simulink model "PreCondition"  (R2018b)
settings: Solver=FixedStepDiscrete  StartTime=0.0  StopTime=10.0  FixedStep=0.01  RelTol=1e-3
undefined symbols (not defined in the file or in its folder): EnergyMgLdShdRq1, HMI_2L_StMd10_Config_Val, HMI_2L_StMd11_Config_Val, HMI_2L_StMd12_Config_Val, HMI_2L_StMd13_Config_Val, HMI_2L_StMd14_Config_Val, HMI_2L_StMd15_Config_Val, HMI_2L_StMd16_Config_Val, HMI_2L_StMd17_Config_Val, HMI_2L_StMd18_Config_Val, HMI_2L_StMd19_Config_Val, HMI_2L_StMd1_Config_Val, HMI_2L_StMd20_Config_Val, HMI_2L_StMd21_Config_Val, HMI_2L_StMd22_Config_Val, HMI_2L_StMd23_Config_Val, HMI_2L_StMd24_Config_Val, HMI_2L_StMd25_Config_Val, HMI_2L_StMd26_Config_Val, HMI_2L_StMd27_Config_Val, HMI_2L_StMd28_Config_Val, HMI_2L_StMd29_Config_Val, HMI_2L_StMd2_Config_Val, HMI_2L_StMd30_Config_Val, HMI_2L_StMd31_Config_Val, HMI_2L_StMd32_Config_Val, HMI_2L_StMd3_Config_Val, HMI_2L_StMd4_Config_Val, HMI_2L_StMd5_Config_Val, HMI_2L_StMd6_Config_Val, HMI_2L_StMd7_Config_Val, HMI_2L_StMd8_Config_Val, HMI_2L_StMd9_Config_Val, HMI_2R_StMd10_Config_Val, HMI_2R_StMd11_Config_Val, HMI_2R_StMd12_Config_Val, HMI_2R_StMd13_Config_Val, HMI_2R_StMd14_Config_Val, HMI_2R_StMd15_Config_Val, HMI_2R_StMd16_Config_Val, HMI_2R_StMd17_Config_Val, HMI_2R_StMd18_Config_Val, HMI_2R_StMd19_Config_Val, HMI_2R_StMd1_Config_Val, HMI_2R_StMd20_Config_Val, HMI_2R_StMd21_Config_Val, HMI_2R_StMd22_Config_Val, HMI_2R_StMd23_Config_Val, HMI_2R_StMd24_Config_Val, HMI_2R_StMd25_Config_Val, HMI_2R_StMd26_Config_Val, HMI_2R_StMd27_Config_Val, HMI_2R_StMd28_Config_Val, HMI_2R_StMd29_Config_Val, HMI_2R_StMd2_Config_Val, HMI_2R_StMd30_Config_Val, HMI_2R_StMd31_Config_Val, HMI_2R_StMd32_Config_Val, HMI_2R_StMd3_Config_Val, HMI_2R_StMd4_Config_Val ... (+94)
(part 4 of 6)

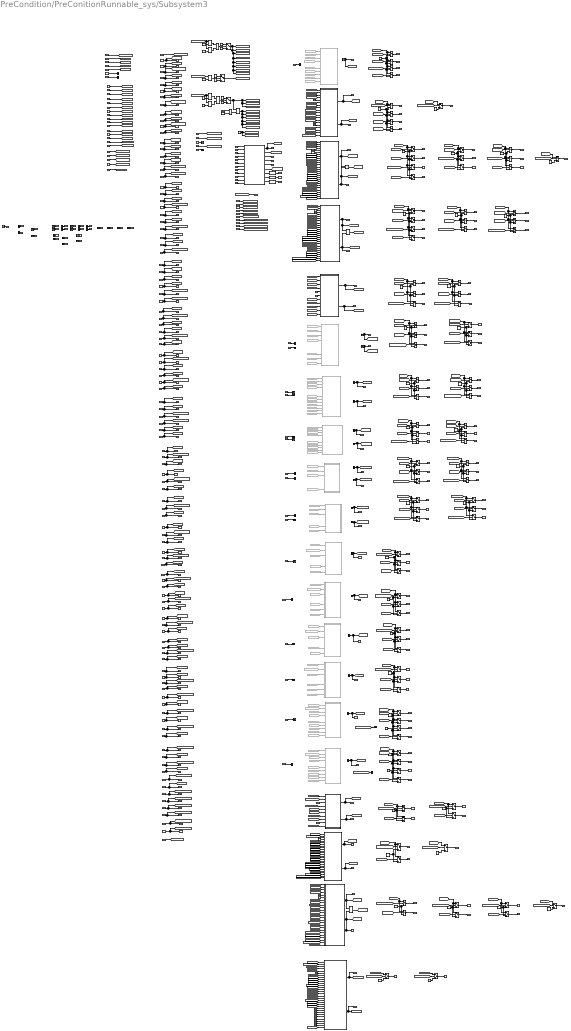
== system PreCondition/PreConitionRunnable_sys/Subsystem3 ==
  note: #大四座的前提条件和AcsEntry一致
  note: NOTE:
      | 2023-08-01:
      | 1.新增mode21~26的前提条件更改，REQ_MSM_778
      | 2.增加PSM,vip或者全躺模式/腿托一键打开增加位置前后判断，REQ_MSM_631/787/788
      | 2023-11-27：
      | 1.腿托一键打开，VIP功能，全躺功能不限制座椅前后位置
      | 2.增加诊断C02C
  note: 4座不包含亲密模式，照看模式
  note: #LyingR
  note: #LyingL
  note: #RcvyR
  note: #VipR
  note: #RcvyL
  note: #VIpL
  note: #LuggageR
  note: #LuggageL
  note: #Family—2R
  note: #Intimacy
  note: #Luggage All
  note: #VIP All
  note: //13，14提供给扶手屏
  note: //2，3提供给扶手屏
  note: #Family—2L
  note: #LgrstOpenLt
  note: #LgrstCloseLt
  note: #LgrstOpenRt
  note: #LgrstCloseRt
  note: #VIPAllOut
  note: #ExVIPR的前提条件和VIPR一致
  SysPwrMd : Inport
  SysPwrMdV : Inport  Port=2
  VoltSts : Inport  Port=3
  EnergyMgLdShdRq : Inport  Port=4
  MmryRclImpctDisRq : Inport  Port=5
  AbgDplyBckp : Inport  Port=6
  AbgDplyBckpV : Inport  Port=7
  VehMovState : Inport  Port=8
  VehSpdAvgDrvnV : Inport  Port=9
  VehSpdAvgDrvn : Inport  Port=10
  DrvStPosRclRspStat : Inport  Port=11
  PassStPosRclRspStat : Inport  Port=12
  SecRwLtStPosRclRspStat : Inport  Port=13
  SecRwRtStPosRclRspStat : Inport  Port=14
  ThdRwLtStPosRclRspStat : Inport  Port=15
  ThdRwRtStPosRclRspStat : Inport  Port=16
  AcsEntryPosLrnd : Inport  Port=17
  AcsExitPosLrnd : Inport  Port=18
  VIPLtPosLrnd : Inport  Port=19
  VIPRtPosLrnd : Inport  Port=20
  LugLtPosLrnd : Inport  Port=21
  LugRtPosLrnd : Inport  Port=22
  RcvyLtPosLrnd : Inport  Port=23
  RcvyRtPosLrnd : Inport  Port=24
  ThdRwLtStOccStatMSMSrc : Inport  Port=25
  ThdRwCtStOccStatMSMSrc : Inport  Port=26
  ThdRwRtStOccStatMSMSrc : Inport  Port=27
  SecRwLtStChldLkReq : Inport  Port=28
  SecRwRtStChldLkReq : Inport  Port=29
  IsDrvStSwAct : Inport  Port=30
  IsPasStSwAct : Inport  Port=31
  Is2LStSwAct : Inport  Port=32
  Is2RStSwAct : Inport  Port=33
  Is3LStSwAct : Inport  Port=34
  Is3RStSwAct : Inport  Port=35
  VeSignalLost2R_463_2L : Inport  Port=36
  VeSignalLost3L_468_2L : Inport  Port=37
  "VeSignalLost3R_46C_2L " : Inport  Port=38
  VeSignalLostCODR_470_2L : Inport  Port=39
  VeSignalLostDR_213_2L : Inport  Port=40
  KeSMSbRoofSWEnable : Inport  Port=41
  VeSignalLostSDM_195_2L : Inport  Port=42
  VeSignalLostFireWall_1D2_2L : Inport  Port=43
  IntimacyLPosLrnd : Inport  Port=44
  IntimacyRPosLrnd : Inport  Port=45
  FamilyLtPosLrnd : Inport  Port=46
  FamilyRtPosLrnd : Inport  Port=47
  LyingLtPosLrnd : Inport  Port=48
  LyingRtPosLrnd : Inport  Port=49
  HMI_2L_StMd1_Config : Inport  Port=50
  HMI_2R_StMd1_Config : Inport  Port=51
  StPassCmprtMdCtrl_Md1_VCUConfig : Inport  Port=52
  StSrv_StMd1_Config : Inport  Port=53
  HMI_2L_StMd2_Config : Inport  Port=54
  HMI_2R_StMd2_Config : Inport  Port=55
  StPassCmprtMdCtrl_Md2_VCUConfig : Inport  Port=56
  StSrv_StMd2_Config : Inport  Port=57
  HMI_2L_StMd10_Config : Inport  Port=58
  HMI_2R_StMd12_Config : Inport  Port=59
  StSrv_StMd10_Config : Inport  Port=60
  StSrv_StMd12_Config : Inport  Port=61
  StPassCmprtMdCtrl_Md10_VCUConfig : Inport  Port=62
  StPassCmprtMdCtrl_Md12_VCUConfig : Inport  Port=63
  HMI_2L_StMd4_Config : Inport  Port=64
  HMI_2R_StMd4_Config : Inport  Port=65
  StSrv_StMd4_Config : Inport  Port=66
  StPassCmprtMdCtrl_Md4_VCUConfig : Inport  Port=67
  HMI_2L_StMd3_Config : Inport  Port=68
  HMI_2R_StMd3_Config : Inport  Port=69
  StSrv_StMd3_Config : Inport  Port=70
  StPassCmprtMdCtrl_Md3_VCUConfig : Inport  Port=71
  HMI_2L_StMd8_Config : Inport  Port=72
  HMI_2R_StMd9_Config : Inport  Port=73
  StSrv_StMd8_Config : Inport  Port=74
  StPassCmprtMdCtrl_Md8_VCUConfig : Inport  Port=75
  StSrv_StMd9_Config : Inport  Port=76
  StPassCmprtMdCtrl_Md9_VCUConfig : Inport  Port=77
  HMI_2L_StMd11_Config : Inport  Port=78
  HMI_2R_StMd13_Config : Inport  Port=79
  StSrv_StMd11_Config : Inport  Port=80
  StSrv_StMd13_Config : Inport  Port=81
  StPassCmprtMdCtrl_Md11_VCUConfig : Inport  Port=82
  StPassCmprtMdCtrl_Md13_VCUConfig : Inport  Port=83
  HMI_2L_StMd5_Config : Inport  Port=84
  HMI_2R_StMd20_Config : Inport  Port=85
  StPassCmprtMdCtrl_Md5_VCUConfig : Inport  Port=86
  StPassCmprtMdCtrl_Md20_VCUConfig : Inport  Port=87
  StSrv_StMd5_Config : Inport  Port=88
  StSrv_StMd20_Config : Inport  Port=89
  HMI_2R_StMd6_Config : Inport  Port=90
  HMI_2L_StMd7_Config : Inport  Port=91
  StPassCmprtMdCtrl_Md6_VCUConfig : Inport  Port=92
  StSrv_StMd6_Config : Inport  Port=93
  StPassCmprtMdCtrl_Md7_VCUConfig : Inport  Port=94
  StSrv_StMd7_Config : Inport  Port=95
  HMI_2L_StMd14_Config : Inport  Port=96
  HMI_2R_StMd15_Config : Inport  Port=97
  StPassCmprtMdCtrl_Md14_VCUConfig : Inport  Port=98
  StPassCmprtMdCtrl_Md15_VCUConfig : Inport  Port=99
  StSrv_StMd14_Config : Inport  Port=100
  StSrv_StMd15_Config : Inport  Port=101
  LgrstOpenLtPosLrnd : Inport  Port=102
  LgrstCloseLtPosLrnd : Inport  Port=103
  LgrstOpenRtPosLrnd : Inport  Port=104
  LgrstCloseRtPosLrnd : Inport  Port=105
  HMI_2L_StMd16_Config : Inport  Port=106
  StPassCmprtMdCtrl_Md16_VCUConfig : Inport  Port=107
  StSrv_StMd16_Config : Inport  Port=108
  HMI_2L_StMd17_Config : Inport  Port=109
  StPassCmprtMdCtrl_Md17_VCUConfig : Inport  Port=110
  StSrv_StMd17_Config : Inport  Port=111
  HMI_2R_StMd18_Config : Inport  Port=112
  StPassCmprtMdCtrl_Md18_VCUConfig : Inport  Port=113
  StSrv_StMd18_Config : Inport  Port=114
  HMI_2R_StMd19_Config : Inport  Port=115
  StPassCmprtMdCtrl_Md19_VCUConfig : Inport  Port=116
  StSrv_StMd19_Config : Inport  Port=117
  IfVeSMSeStNumConfig : Inport  Port=118
  KeSMSLegrstDisFwdBkwdPos : Inport  Port=119
  SecRwLtStFrwdBkwdPos : Inport  Port=120
  "SecRwLtStFrwdBkwdPosV " : Inport  Port=121
  "SecRwRtStFrwdBkwdPos " : Inport  Port=122
  "SecRwRtStFrwdBkwdPosV " : Inport  Port=123
  AcsEntry4s2LPosLrnd : Inport  Port=124
  HMI_2L_StMd21_Config : Inport  Port=125
  StPassCmprtMdCtrl_Md21_VCUConfig : Inport  Port=126
  StSrv_StMd21_Config : Inport  Port=127
  AcsEntry4s2RPosLrnd : Inport  Port=128
  HMI_2R_StMd23_Config : Inport  Port=129
  StPassCmprtMdCtrl_Md23_VCUConfig : Inport  Port=130
  StSrv_StMd23_Config : Inport  Port=131
  AcsExit4s2LPosLrnd : Inport  Port=132
  HMI_2L_StMd22_Config : Inport  Port=133
  StPassCmprtMdCtrl_Md22_VCUConfig : Inport  Port=134
  StSrv_StMd22_Config : Inport  Port=135
  AcsExit4s2RPosLrnd : Inport  Port=136
  HMI_2R_StMd24_Config : Inport  Port=137
  StPassCmprtMdCtrl_Md24_VCUConfig : Inport  Port=138
  StSrv_StMd24_Config : Inport  Port=139
  AcsEntryAll4sFwdPosLrnd : Inport  Port=140
  HMI_2L_StMd26_Config : Inport  Port=141
  HMI_2R_StMd26_Config : Inport  Port=142
  StPassCmprtMdCtrl_Md26_VCUConfig : Inport  Port=143
  StSrv_StMd26_Config : Inport  Port=144
  AcsEntryAll4sBwdPosLrnd : Inport  Port=145
  HMI_2L_StMd25_Config : Inport  Port=146
  HMI_2R_StMd25_Config : Inport  Port=147
  StPassCmprtMdCtrl_Md25_VCUConfig : Inport  Port=148
  StSrv_StMd25_Config : Inport  Port=149
  IfKeSMSbSeatMovFrwdBkwdEnable : Inport  Port=150
  PassReclinerPosLrnd : Inport  Port=151
  unfold3LPosLrnd : Inport  Port=152
  unfold3RPosLrnd : Inport  Port=153
  NotCoDrvStOccStatBDFSrc : Inport  Port=154
  StPassCmprtMdCtrl_Md30_VCUConfig : Inport  Port=155
  StSrv_StMd30_Config : Inport  Port=156
  StPassCmprtMdCtrl_Md31_VCUConfig : Inport  Port=157
  StSrv_StMd31_Config : Inport  Port=158
  StPassCmprtMdCtrl_Md32_VCUConfig : Inport  Port=159
  StSrv_StMd32_Config : Inport  Port=160
  VIPLtOutPosLrnd : Inport  Port=161
  VIPRtOutPosLrnd : Inport  Port=162
  StPassCmprtMdCtrl_Md27_VCUConfig : Inport  Port=163
  StSrv_StMd27_Config : Inport  Port=164
  StPassCmprtMdCtrl_Md28_VCUConfig : Inport  Port=165
  StSrv_StMd28_Config : Inport  Port=166
  StPassCmprtMdCtrl_Md29_VCUConfig : Inport  Port=167
  StSrv_StMd29_Config : Inport  Port=168
  ThdRwLtStCshnFldUpwdDnwdPos : Inport  Port=169
  ThdRwLtStCshnFldUpwdDnwdPosV : Inport  Port=170
  ThdRwRtStCshnFldUpwdDnwdPos : Inport  Port=171
  ThdRwRtStCshnFldUpwdDnwdPosV : Inport  Port=172
  ThdRwLtStChldLkReq : Inport  Port=173
  NotSecRowLeStOccStatBDFSrc : Inport  Port=174
  NotSecRowRtStOccStatBDFSrc : Inport  Port=175
  SecRwLtStBkReclnUpwdDnwdPos : Inport  Port=176
  SecRwLtStBkReclnUpwdDnwdPosV : Inport  Port=177
  SecRwRtStBkReclnUpwdDnwdPos : Inport  Port=178
  SecRwRtStBkReclnUpwdDnwdPosV : Inport  Port=179
  KeSMSuSecRwStBackPosDelta : Inport  Port=180
  StPassCmprtMdCtrl_Md53_VCUConfig : Inport  Port=181
  StPassCmprtMdCtrl_Md56_VCUConfig : Inport  Port=182
  KeSMSuThrdRwCushFoldPosThreshold : Inport  Port=183
  StPassCmprtMdCtrl_Md57_VCUConfig : Inport  Port=184
  StPassCmprtMdCtrl_Md58_VCUConfig : Inport  Port=185
  PasReclinerPosAvail : Inport  Port=186
  KeSMSwAcsMd32SecRwLtStBkReclnUpwdDnwdPos1 : Inport  Port=187
  KeSMSwAcsMd53SecRwRtStBkReclnUpwdDnwdPos1 : Inport  Port=188
  KeSMSwAcsMd8SecRwLtStBkReclnUpwdDnwdPos : Inport  Port=189
  KeSMSwAcsMd9SecRwRtStBkReclnUpwdDnwdPos : Inport  Port=190
  WholeVehMemPosLrnd : Inport  Port=191
  StPassCmprtMdCtrl_Md61_VCUConfig : Inport  Port=192
  StPassCmprtMdCtrl_Md62_VCUConfig : Inport  Port=193
  KeSMSwSeatBkLimitPos : Inport  Port=194
  KeSMSwSeatBkLimitPosDelt : Inport  Port=195
  Md61PassStBkReclnTrgtPos : Inport  Port=196
  Md61ThdRwLtStCshnFldUpwdDnwdTrgtPos : Inport  Port=197
  Md61ThdRwRtStCshnFldUpwdDnwdTrgtPos : Inport  Port=198
  Md62PassStBkReclnTrgtPos : Inport  Port=199
  Md62ThdRwLtStCshnFldUpwdDnwdTrgtPos : Inport  Port=200
  Md62ThdRwRtStCshnFldUpwdDnwdTrgtPos : Inport  Port=201
  KeSMSuThrdRwCushFoldPosDelta : Inport  Port=202
  AND{,1..3,5} (5 alike) : Logic  Operator=OR  AllPortsSameDT=off  OutDataTypeStr=boolean
  AND4 : Logic  AllPortsSameDT=off  OutDataTypeStr=boolean
  AcsEntry4s2LMd : Subsystem  Commented=on
  AcsEntry4s2RMd : Subsystem  Commented=on
  AcsEntryAll4sBwdMd : Subsystem  Commented=on
  AcsEntryAll4sFwdMd : Subsystem  Commented=on
  AcsEntyAvl : Subsystem
  AcsExit4s2LMd : Subsystem  Commented=on
  AcsExit4s2RMd : Subsystem  Commented=on
  AcsExtAvl : Subsystem  Commented=on
  "CommCond " : Subsystem
  Constant : Constant  Value=IfVeSMSeStNumConfig.SeatNum7Config  OutDataTypeStr=Enum: IfVeSMSeStNumConfig
  Constant1 : Constant  Value=IfVeSMSeStNumConfig.SeatNum6Config  OutDataTypeStr=Enum: IfVeSMSeStNumConfig
  Constant{3,8..34,38..45,48..52} (41 alike) : Constant  Value=0  OutDataTypeStr=boolean
  Constant{2,4,7,47} (4 alike) : Constant  OutDataTypeStr=boolean
  Constant35 : Constant  Value=2  OutDataTypeStr=uint8
  Constant36 : Constant  OutDataTypeStr=uint8
  Constant37 : Constant  OutDataTypeStr=uint8
  Constant46 : Constant  Value=IfVeSMSeStNumConfig.SeatNum7Config  OutDataTypeStr=Enum: IfVeSMSeStNumConfig
  Constant5 : Constant  Value=IfVeSMSeStNumConfig.SeatNum4Config  OutDataTypeStr=Enum: IfVeSMSeStNumConfig
  Constant6 : Constant  Value=IfVeSMSeStNumConfig.SeatNum4PConfig  OutDataTypeStr=Enum: IfVeSMSeStNumConfig
  Data Type Conversion : DataTypeConversion  OutDataTypeStr=Enum: DiagAbgDly
  Data Type Conversion1 : DataTypeConversion  OutDataTypeStr=Enum: DiagVehMovState
  Data Type Conversion2 : DataTypeConversion  OutDataTypeStr=Enum: DiagVehSpdAvgDrvn
  Equal{,1..5} (6 alike) : RelationalOperator  Operator===  OutDataTypeStr=boolean  RndMeth=Simplest
  FamilyMd : Subsystem  Commented=on
  From : From  Commented=on  GotoTag=AcsMdExtConfig
  From{100,206..207,239,249} (5 alike) : From  Commented=on  GotoTag=SecRwLtStChldLkReq
  From{101,222,237..238,250} (5 alike) : From  Commented=on  GotoTag=SecRwRtStChldLkReq
  From{49,76,91,102,121,217,232,242,253} (9 alike) : From  Commented=on  GotoTag=VeSignalLost2R_463_2L
  From105 : From  Commented=on  GotoTag=LgrstLtMdConfig
  From{27,56,95,106,113,202..203,223,229..230,248} (11 alike) : From  Commented=on  GotoTag=CommCond
  From{2,17,31,53,58,96,107,278,295} (9 alike) : From  Commented=on  GotoTag=SecRwLtStPosRclRspStat
  From108 : From  Commented=on  GotoTag=LgrstRtMdConfig
  From{43,60,62,98,109,209,224,241,251} (9 alike) : From  Commented=on  GotoTag=Is2LStSwAct
  From{3,18,42,59,97,115,277,279,296} (9 alike) : From  Commented=on  GotoTag=SecRwRtStPosRclRspStat
  From{48,61,63,99,116,216,231,240,252} (9 alike) : From  Commented=on  GotoTag=Is2RStSwAct
  From14 : From  Commented=on  GotoTag=IsPasStSwAct
  From201 : From  Commented=on  GotoTag=AcsEntry4s2LMdConfig
  From204 : From  Commented=on  GotoTag=AcsEntry4s2RMdConfig
  From205 : From  Commented=on  GotoTag=AcsExit4s2LMdConfig
  From208 : From  Commented=on  GotoTag=AcsExit4s2RMdConfig
  From214 : From  Commented=on  GotoTag=AcsEntryAll4sBwdMdConfig
  From215 : From  Commented=on  GotoTag=AcsEntryAll4sFwdMdConfig
  From30 : From  Commented=on  GotoTag=IntimacyMdConfig
  From4 : From  Commented=on  GotoTag=CommCondWithSpeed
  From57 : From  Commented=on  GotoTag=FamilyMdConfig
  From64 : From  Commented=on  GotoTag=Is3RStSwAct
  From9 : From  Commented=on  GotoTag=IsDrvStSwAct
  From90 : From  Commented=on  GotoTag=Is3LStSwAct
  From92 : From  Commented=on  GotoTag=VeSignalLost3L_468_2L
  From93 : From  Commented=on  GotoTag=VeSignalLost3R_46C_2L
  From94 : From  Commented=on  GotoTag=LyingMdConfig
  Ground{,1..41} (42 alike) : Ground
  IntimacyMd : Subsystem  Commented=on
  LgrstOpenLtMd : Subsystem  Commented=on
  LgrstOpenRtMd : Subsystem  Commented=on
  LugMdAvl : Subsystem
  LyingMd : Subsystem  Commented=on
  PasReclinerMd : Subsystem
  RcvyMdAvl : Subsystem
  Switch{,1..104} (105 alike) : Switch  Criteria=u2 > Threshold
  Terminator : Terminator
  Terminator1 : Terminator
  Terminator_{1..20,75} (21 alike) : Terminator
  VipMdAvl : Subsystem
  VipOutMdAvl : Subsystem
  WholeVehMem : Subsystem
  unfoldMd : Subsystem
  CommCond : Outport
  CommExitCondwithSpeed : Outport  Port=2
  CommExitCond : Outport  Port=3
  PwrMdChked : Outport  Port=4
  HMIMd1Cfg_2L : Outport  Port=5
  HMIMd1Cfg_2R : Outport  Port=6
  HMIMd1Avl_2L : Outport  Port=7
  HMIMd1Avl_2R : Outport  Port=8
  HMIMd2Cfg_2L : Outport  Port=9
  HMIMd2Cfg_2R : Outport  Port=10
  HMIMd2Avl_2L : Outport  Port=11
  HMIMd2Avl_2R : Outport  Port=12
  HMIMd3Cfg_2L : Outport  Port=13
  HMIMd3Cfg_2R : Outport  Port=14
  HMIMd3Avl_2L : Outport  Port=15
  HMIMd3Avl_2R : Outport  Port=16
  HMIMd4Cfg_2L : Outport  Port=17
  HMIMd4Cfg_2R : Outport  Port=18
  HMIMd4Avl_2L : Outport  Port=19
  HMIMd4Avl_2R : Outport  Port=20
  HMIMd6Cfg_2L : Outport  Port=21
  HMIMd6Avl_2L : Outport  Port=22
  HMIMd7Cfg_2R : Outport  Port=23
  HMIMd7Avl_2R : Outport  Port=24
  HMIMd8Cfg_2L : Outport  Port=25
  HMIMd8Cfg_2R : Outport  Port=26
  HMIMd8Avl_2L : Outport  Port=27
  HMIMd8Avl_2R : Outport  Port=28
  HMIMd9Cfg_2L : Outport  Port=29
  HMIMd9Cfg_2R : Outport  Port=30
  HMIMd9Avl_2L : Outport  Port=31
  HMIMd9Avl_2R : Outport  Port=32
  HMIMd10Cfg_2L : Outport  Port=33
  HMIMd10Cfg_2R : Outport  Port=34
  HMIMd10Avl_2L : Outport  Port=35
  HMIMd10Avl_2R : Outport  Port=36
  HMIMd11Cfg_2L : Outport  Port=37
  HMIMd11Cfg_2R : Outport  Port=38
  HMIMd11Avl_2L : Outport  Port=39
  HMIMd11Avl_2R : Outport  Port=40
  HMIMd12Cfg_2L : Outport  Port=41
  HMIMd12Cfg_2R : Outport  Port=42
  HMIMd12Avl_2L : Outport  Port=43
  HMIMd12Avl_2R : Outport  Port=44
  HMIMd13Cfg_2L : Outport  Port=45
  HMIMd13Cfg_2R : Outport  Port=46
  HMIMd13Avl_2L : Outport  Port=47
  HMIMd13Avl_2R : Outport  Port=48
  HMIMd14Cfg_2L : Outport  Port=49
  HMIMd14Cfg_2R : Outport  Port=50
  HMIMd14Avl_2R : Outport  Port=51
  HMIMd15Cfg_2L : Outport  Port=52
  HMIMd15Cfg_2R : Outport  Port=53
  HMIMd15Avl_2L : Outport  Port=54
  StPassCmprtMdCtrl_Md1_VCUAvl : Outport  Port=55
  StPassCmprtMdCtrl_Md2_VCUAvl : Outport  Port=56
  StPassCmprtMdCtrl_Md3_VCUAvl : Outport  Port=57
  StPassCmprtMdCtrl_Md4_VCUAvl : Outport  Port=58
  StPassCmprtMdCtrl_Md8_VCUAvl : Outport  Port=59
  StPassCmprtMdCtrl_Md9_VCUAvl : Outport  Port=60
  StPassCmprtMdCtrl_Md10_VCUAvl : Outport  Port=61
  StPassCmprtMdCtrl_Md11_VCUAvl : Outport  Port=62
  StPassCmprtMdCtrl_Md12_VCUAvl : Outport  Port=63
  StPassCmprtMdCtrl_Md13_VCUAvl : Outport  Port=64
  StPassCmprtMdCtrl_Md1_VCUCfg : Outport  Port=65
  StPassCmprtMdCtrl_Md2_VCUCfg : Outport  Port=66
  StPassCmprtMdCtrl_Md3_VCUCfg : Outport  Port=67
  StPassCmprtMdCtrl_Md4_VCUCfg : Outport  Port=68
  StPassCmprtMdCtrl_Md8_VCUCfg : Outport  Port=69
  StPassCmprtMdCtrl_Md9_VCUCfg : Outport  Port=70
  StPassCmprtMdCtrl_Md10_VCUCfg : Outport  Port=71
  StPassCmprtMdCtrl_Md11_VCUCfg : Outport  Port=72
  StPassCmprtMdCtrl_Md12_VCUCfg : Outport  Port=73
  StPassCmprtMdCtrl_Md13_VCUCfg : Outport  Port=74
  StPassCmprtMdCtrl_Md14_VCUCfg : Outport  Port=75
  StPassCmprtMdCtrl_Md15_VCUCfg : Outport  Port=76
  StSrvCfg_Md1 : Outport  Port=77
  StSrvCfg_Md2 : Outport  Port=78
  StSrvCfg_Md3 : Outport  Port=79
  StSrvCfg_Md4 : Outport  Port=80
  StSrvCfg_Md8 : Outport  Port=81
  StSrvCfg_Md9 : Outport  Port=82
  StSrvCfg_Md10 : Outport  Port=83
  StSrvCfg_Md11 : Outport  Port=84
  StSrvCfg_Md12 : Outport  Port=85
  StSrvCfg_Md13 : Outport  Port=86
  StSrvCfg_Md14 : Outport  Port=87
  StSrvCfg_Md15 : Outport  Port=88
  StSrvAvl_Md1 : Outport  Port=89
  StSrvAvl_Md2 : Outport  Port=90
  StSrvAvl_Md3 : Outport  Port=91
  StSrvAvl_Md4 : Outport  Port=92
  StSrvAvl_Md8 : Outport  Port=93
  StSrvAvl_Md9 : Outport  Port=94
  StSrvAvl_Md10 : Outport  Port=95
  StSrvAvl_Md11 : Outport  Port=96
  StSrvAvl_Md12 : Outport  Port=97
  StSrvAvl_Md13 : Outport  Port=98
  StPassCmprtMdRfCtrlSwCstStAvl : Outport  Port=99
  AcsMdEntyAvl : Outport  Port=100
  AcsMdExtAvl : Outport  Port=101
  "VipMdLtAvl " : Outport  Port=102
  VipMdRtAvl : Outport  Port=103
  LugMdLtAvl : Outport  Port=104
  LugMdRtAvl : Outport  Port=105
  RcvyMdLtAvl : Outport  Port=106
  RcvyMdRtAvl : Outport  Port=107
  IntimacyLMdAvl : Outport  Port=108
  IntimacyRMdAvl : Outport  Port=109
  FamilyMdLtAvl : Outport  Port=110
  FamilyMdRtAvl : Outport  Port=111
  LyingMdLtAvl : Outport  Port=112
  LyingMdRtAvl : Outport  Port=113
  HMIMd5Cfg_2L : Outport  Port=114
  HMIMd20Cfg_2R : Outport  Port=115
  HMIMd5Cfg_2R : Outport  Port=116
  StPassCmprtMdCtrl_Md5_VCUCfg : Outport  Port=117
  StPassCmprtMdCtrl_Md20_VCUCfg : Outport  Port=118
  StSrvCfg_Md5 : Outport  Port=119
  StSrvCfg_Md20 : Outport  Port=120
  HMIMd6Cfg_2R : Outport  Port=121
  HMIMd7Cfg_2L : Outport  Port=122
  StPassCmprtMdCtrl_Md6_VCUCfg : Outport  Port=123
  StPassCmprtMdCtrl_Md7_VCUCfg : Outport  Port=124
  StSrvCfg_Md6 : Outport  Port=125
  StSrvCfg_Md7 : Outport  Port=126
  HMIMd5Avl_2L : Outport  Port=127
  HMIMd20Avl_2R : Outport  Port=128
  StPassCmprtMdCtrl_Md5_VCUAvl : Outport  Port=129
  StSrvAvl_Md5 : Outport  Port=130
  HMIMd6Avl_2R : Outport  Port=131
  StPassCmprtMdCtrl_Md6_VCUAvl : Outport  Port=132
  StSrvAvl_Md6 : Outport  Port=133
  HMIMd7Avl_2L : Outport  Port=134
  StPassCmprtMdCtrl_Md7_VCUAvl : Outport  Port=135
  StSrvAvl_Md7 : Outport  Port=136
  HMIMd14Avl_2L : Outport  Port=137
  StPassCmprtMdCtrl_Md14_VCUAvl : Outport  Port=138
  StSrvAvl_Md14 : Outport  Port=139
  HMIMd15Avl_2R : Outport  Port=140
  StPassCmprtMdCtrl_Md15_VCUAvl : Outport  Port=141
  StSrvAvl_Md15 : Outport  Port=142
  DiagAbgDly : Outport  Port=143
  DiagVehMovState : Outport  Port=144
  DiagVehSpdAvgDrvn : Outport  Port=145
  LgrstOpenLtMdAvl : Outport  Port=146
  HMIMd16Cfg_2L : Outport  Port=147
  HMIMd16Cfg_2R : Outport  Port=148
  StPassCmprtMdCtrl_Md16_VCUCfg : Outport  Port=149
  StSrvCfg_Md16 : Outport  Port=150
  HMIMd16Avl_2L : Outport  Port=151
  StPassCmprtMdCtrl_Md16_VCUAvl : Outport  Port=152
  StSrvAvl_Md16 : Outport  Port=153
  HMIMd17Cfg_2R : Outport  Port=154
  HMIMd17Cfg_2L : Outport  Port=155
  StPassCmprtMdCtrl_Md17_VCUCfg : Outport  Port=156
  StSrvCfg_Md17 : Outport  Port=157
  LgrstCloseLtMdAvl : Outport  Port=158
  HMIMd17Avl_2L : Outport  Port=159
  StPassCmprtMdCtrl_Md17_VCUAvl : Outport  Port=160
  StSrvAvl_Md17 : Outport  Port=161
  HMIMd18Cfg_2L : Outport  Port=162
  HMIMd19Cfg_2L : Outport  Port=163
  HMIMd18Cfg_2R : Outport  Port=164
  StPassCmprtMdCtrl_Md18_VCUCfg : Outport  Port=165
  StSrvCfg_Md18 : Outport  Port=166
  HMIMd19Cfg_2R : Outport  Port=167
  StPassCmprtMdCtrl_Md19_VCUCfg : Outport  Port=168
  StSrvCfg_Md19 : Outport  Port=169
  LgrstOpenRtMdAvl : Outport  Port=170
  HMIMd18Avl_2R : Outport  Port=171
  StPassCmprtMdCtrl_Md18_VCUAvl : Outport  Port=172
  StSrvAvl_Md18 : Outport  Port=173
  LgrstCloseRtMdAvl : Outport  Port=174
  HMIMd19Avl_2R : Outport  Port=175
  StPassCmprtMdCtrl_Md19_VCUAvl : Outport  Port=176
  StSrvAvl_Md19 : Outport  Port=177
  StPassCmprtMdCtrl_Md20_VCUAvl : Outport  Port=178
  StSrvAvl_Md20 : Outport  Port=179
  AcsEntry4s2LAvl : Outport  Port=180
  HMIMd21Avl_2L : Outport  Port=181
  StPassCmprtMdCtrl_Md21_VCUAvl : Outport  Port=182
  StSrvAvl_Md21 : Outport  Port=183
  HMIMd21Cfg_2L : Outport  Port=184
  StPassCmprtMdCtrl_Md21_VCUCfg : Outport  Port=185
  StSrvCfg_Md21 : Outport  Port=186
  AcsEntry4s2RAvl : Outport  Port=187
  HMIMd23Cfg_2R : Outport  Port=188
  StPassCmprtMdCtrl_Md23_VCUCfg : Outport  Port=189
  StSrvCfg_Md23 : Outport  Port=190
  StPassCmprtMdCtrl_Md23_VCUAvl : Outport  Port=191
  HMIMd23Avl_2R : Outport  Port=192
  StSrvAvl_Md23 : Outport  Port=193
  AcsExit4s2LAvl : Outport  Port=194
  HMIMd22Cfg_2L : Outport  Port=195
  StPassCmprtMdCtrl_Md22_VCUCfg : Outport  Port=196
  StSrvCfg_Md22 : Outport  Port=197
  StPassCmprtMdCtrl_Md22_VCUAvl : Outport  Port=198
  HMIMd22Avl_2L : Outport  Port=199
  StSrvAvl_Md22 : Outport  Port=200
  AcsExit4s2RAvl : Outport  Port=201
  HMIMd24Cfg_2R : Outport  Port=202
  StPassCmprtMdCtrl_Md24_VCUCfg : Outport  Port=203
  StSrvCfg_Md24 : Outport  Port=204
  StPassCmprtMdCtrl_Md24_VCUAvl : Outport  Port=205
  HMIMd24Avl_2R : Outport  Port=206
  StSrvAvl_Md24 : Outport  Port=207
  AcsEntryAll4sFwdAvl : Outport  Port=208
  HMIMd26Cfg_2L : Outport  Port=209
  HMIMd26Cfg_2R : Outport  Port=210
  StPassCmprtMdCtrl_Md26_VCUCfg : Outport  Port=211
  StSrvCfg_Md26 : Outport  Port=212
  HMIMd26Avl_2L : Outport  Port=213
  HMIMd26Avl_2R : Outport  Port=214
  StPassCmprtMdCtrl_Md26_VCUAvl : Outport  Port=215
  StSrvAvl_Md26 : Outport  Port=216
  AcsEntryAll4sBwdAvl : Outport  Port=217
  HMIMd25Cfg_2L : Outport  Port=218
  HMIMd25Cfg_2R : Outport  Port=219
  StPassCmprtMdCtrl_Md25_VCUCfg : Outport  Port=220
  StSrvCfg_Md25 : Outport  Port=221
  HMIMd25Avl_2L : Outport  Port=222
  HMIMd25Avl_2R : Outport  Port=223
  StPassCmprtMdCtrl_Md25_VCUAvl : Outport  Port=224
  StSrvAvl_Md25 : Outport  Port=225
  "PasReclinerAvl " : Outport  Port=226
  StPassCmprtMdCtrl_Md30_VCUCfg : Outport  Port=227
  StSrvCfg_Md30 : Outport  Port=228
  StPassCmprtMdCtrl_Md31_VCUCfg : Outport  Port=229
  StSrvCfg_Md31 : Outport  Port=230
  StPassCmprtMdCtrl_Md30_VCUAvl : Outport  Port=231
  StSrvAvl_Md30 : Outport  Port=232
  StPassCmprtMdCtrl_Md31_VCUAvl : Outport  Port=233
  StSrvAvl_Md31 : Outport  Port=234
  unfold3LAvl : Outport  Port=235
  StPassCmprtMdCtrl_Md32_VCUCfg : Outport  Port=236
  StSrvCfg_Md32 : Outport  Port=237
  StPassCmprtMdCtrl_Md32_VCUAvl : Outport  Port=238
  StSrvAvl_Md32 : Outport  Port=239
  unfold3RAvl : Outport  Port=240
  VipLtOutMdAvl : Outport  Port=241
  VipRtOutMdAvl : Outport  Port=242
  StPassCmprtMdCtrl_Md29_VCUAvl : Outport  Port=243
  StPassCmprtMdCtrl_Md27_VCUAvl : Outport  Port=244
  StPassCmprtMdCtrl_Md28_VCUAvl : Outport  Port=245
  StSrvAvl_Md29 : Outport  Port=246
  StSrvAvl_Md27 : Outport  Port=247
  StSrvAvl_Md28 : Outport  Port=248
  StPassCmprtMdCtrl_Md27_VCUCfg : Outport  Port=249
  StSrvCfg_Md27 : Outport  Port=250
  StPassCmprtMdCtrl_Md28_VCUCfg : Outport  Port=251
  StSrvCfg_Md28 : Outport  Port=252
  StPassCmprtMdCtrl_Md29_VCUCfg : Outport  Port=253
  StSrvCfg_Md29 : Outport  Port=254
  PasReclinerExitAvl : Outport  Port=255
  StPassCmprtMdCtrl_Md53_VCUCfg : Outport  Port=256
  StPassCmprtMdCtrl_Md53_VCUAvl : Outport  Port=257
  StPassCmprtMdCtrl_Md56_VCUCfg : Outport  Port=258
  StPassCmprtMdCtrl_Md56_VCUAvl : Outport  Port=259
  StPassCmprtMdCtrl_Md57_VCUCfg : Outport  Port=260
  StPassCmprtMdCtrl_Md58_VCUCfg : Outport  Port=261
  StPassCmprtMdCtrl_Md57_VCUAvl : Outport  Port=262
  StPassCmprtMdCtrl_Md58_VCUAvl : Outport  Port=263
  Big4SeatAvl : Outport  Port=264
  StPassCmprtMdCtrl_Md61_VCUAvl : Outport  Port=265
  StPassCmprtMdCtrl_Md62_VCUAvl : Outport  Port=266
  M61WholeVehMemAvl : Outport  Port=267
  M62WholeVehMemAvl : Outport  Port=268
  StPassCmprtMdCtrl_Md61_VCUCfg : Outport  Port=269
  StPassCmprtMdCtrl_Md62_VCUCfg : Outport  Port=270
  wires:
  From2/1 -> AcsExtAvl/3(SecRwLtStPosRclRspStat)
  VipMdAvl/1(VipMdLtAvl) -> "VipMdLtAvl "/1, [VipMdLtAvl], AND/1
  [LugMdConfig] -> LugMdAvl/2(LugMdConfig)
  "CommCond "/1("CommCond ") -> CommCond/1, [CommCond]
  [SecRwRtStChldLkReq] -> RcvyMdAvl/8(SecRwRtStChldLkReq)
  RcvyMdAvl/1(RcvyMdLtAvl) -> RcvyMdLtAvl/1, [RcvyMdLtAvl]
  [ThdRwCtStOccStat] -> LugMdAvl/6(ThdRwCtStOccStat)
  SecRwLtStChldLkReq/1 -> [SecRwLtStChldLkReq]
  SecRwRtStPosRclRspStat/1 -> [SecRwRtStPosRclRspStat]
  [CommCond] -> RcvyMdAvl/1(CommCond)
  [RcvyMdConfig] -> RcvyMdAvl/2(RcvyMdConfig)
  [CommCond] -> VipMdAvl/1(CommCond)
  RcvyRtPosLrnd/1 -> RcvyMdAvl/6(RcvyRtPosLrnd)
  [ThdRwRtStOccStat] -> LugMdAvl/7(ThdRwRtStOccStat)
  PassStPosRclRspStat/1 -> [PassStPosRclRspStat]
  ThdRwRtStOccStatMSMSrc/1 -> [ThdRwRtStOccStat]
  RcvyMdAvl/2(RcvyMdRtAvl) -> RcvyMdRtAvl/1, [RcvyMdRtAvl]
  ThdRwLtStOccStatMSMSrc/1 -> [ThdRwLtStOccStat]
  LugMdAvl/2(LugMdRtAvl) -> [LugMdRtAvl], LugMdRtAvl/1, AND1/2
  VipMdAvl/2(VipMdRtAvl) -> AND/2, [VipMdRtAvl], VipMdRtAvl/1
  [SecRwRtStPosRclRspStat] -> RcvyMdAvl/4(SecRwRtStPosRclRspStat)
  [ThdRwRtStOccStat] -> VipMdAvl/9(ThdRwRtStOccStat)
  AcsEntyAvl/1("AcsMdEntyAvl ") -> [AcsMdEntyAvl], AcsMdEntyAvl/1
  [VipMdConfig] -> VipMdAvl/2(VipMdConfig)
  [SecRwLtStPosRclRspStat] -> VipMdAvl/3(SecRwLtStPosRclRspStat)
  [SecRwRtStPosRclRspStat] -> VipMdAvl/4(SecRwRtStPosRclRspStat)
  [ThdRwLtStOccStat] -> VipMdAvl/7(ThdRwLtStOccStat)
  SecRwRtStChldLkReq/1 -> [SecRwRtStChldLkReq]
  RcvyLtPosLrnd/1 -> RcvyMdAvl/5(RcvyLtPosLrnd)
  MmryRclImpctDisRq/1 -> "CommCond "/5(MmryRclImpctDisRq)
  [SecRwLtStPosRclRspStat] -> RcvyMdAvl/3(SecRwLtStPosRclRspStat)
  [SecRwLtStChldLkReq] -> VipMdAvl/10(SecRwLtStChldLkReq)
  [SecRwRtStChldLkReq] -> VipMdAvl/11(SecRwRtStChldLkReq)
  [ThdRwCtStOccStat] -> VipMdAvl/8(ThdRwCtStOccStat)
  [SecRwLtStChldLkReq] -> RcvyMdAvl/7(SecRwLtStChldLkReq)
  ThdRwCtStOccStatMSMSrc/1 -> [ThdRwCtStOccStat]
  SysPwrMdV/1 -> "CommCond "/2(SysPwrMdV)
  [CommCondWithSpeed] -> LugMdAvl/1(CommCond)
  [SecRwLtStPosRclRspStat] -> AcsEntyAvl/3(SecRwLtStPosRclRspStat)
  AbgDplyBckp/1 -> "CommCond "/6(AbgDplyBckp)
  DrvStPosRclRspStat/1 -> [DrvStPosRclRspStat]
  From4/1 -> AcsExtAvl/1(CommCond)
  From3/1 -> AcsExtAvl/4(SecRwRtStPosRclRspStat)
  From/1 -> AcsExtAvl/2(AcsMdExitConfig)
  [ThdRwLtStOccStat] -> LugMdAvl/5(ThdRwLtStOccStat)
  SecRwLtStPosRclRspStat/1 -> [SecRwLtStPosRclRspStat]
  ThdRwLtStPosRclRspStat/1 -> Terminator/1
  ThdRwRtStPosRclRspStat/1 -> Terminator1/1
  [SecRwRtStPosRclRspStat] -> AcsEntyAvl/4(SecRwRtStPosRclRspStat)
  [CommCondWithSpeed] -> AcsEntyAvl/1(CommCond)
  [AcsMdEtryConfig] -> AcsEntyAvl/2(AcsMdEtryConfig)
  VoltSts/1 -> "CommCond "/3(VoltSts)
  EnergyMgLdShdRq/1 -> "CommCond "/4(EnergyMgLdShdRq)
  AbgDplyBckpV/1 -> "CommCond "/7(AbgDplyBckpV)
  VehSpdAvgDrvnV/1 -> "CommCond "/9(VehSpdAvgDrvnV)
  VehMovState/1 -> "CommCond "/8(VehMovState)
  VehSpdAvgDrvn/1 -> "CommCond "/10(VehSpdAvgDrvn)
  "CommCond "/3(CommExitCondwithSpeed) -> CommExitCondwithSpeed/1
  "CommCond "/5(PwrMdChked) -> PwrMdChked/1
  "CommCond "/6(isVehStatAndSpeedOK) -> [isVehStatAndSpeedOK]
  "CommCond "/4(CommExitCond) -> CommExitCond/1
  IsDrvStSwAct/1 -> [IsDrvStSwAct]
  IsPasStSwAct/1 -> [IsPasStSwAct]
  Is2LStSwAct/1 -> [Is2LStSwAct]
  Is2RStSwAct/1 -> [Is2RStSwAct]
  Is3LStSwAct/1 -> [Is3LStSwAct]
  Is3RStSwAct/1 -> [Is3RStSwAct]
  From62/1 -> AcsExtAvl/8(Is2LStSwAct)
  From63/1 -> AcsExtAvl/9(Is2RStSwAct)
  [Is2LStSwAct] -> AcsEntyAvl/6(Is2LStSwAct)
  [Is2RStSwAct] -> AcsEntyAvl/7(Is2RStSwAct)
  [Is3RStSwAct] -> AcsEntyAvl/9(Is3RStSwAct)
  [Is2LStSwAct] -> VipMdAvl/14(Is2LStSwAct)
  [Is3LStSwAct] -> VipMdAvl/16(Is3LStSwAct)
  [Is3RStSwAct] -> VipMdAvl/17(Is3RStSwAct)
  [Is3LStSwAct] -> LugMdAvl/8(Is3LStSwAct)
  [Is3RStSwAct] -> LugMdAvl/9(Is3RStSwAct)
  [Is2LStSwAct] -> RcvyMdAvl/9(Is2LStSwAct)
  [Is2RStSwAct] -> RcvyMdAvl/10(Is2RStSwAct)
  [IfVeSMSeStNumConfig] -> VipMdAvl/18(IfVeSMSeStNumConfig)
  [IfVeSMSeStNumConfig] -> LugMdAvl/12(IfVeSMSeStNumConfig)
  VeSignalLost2R_463_2L/1 -> [VeSignalLost2R_463_2L]
  "VeSignalLost3R_46C_2L "/1 -> [VeSignalLost3R_46C_2L]
  VeSignalLostCODR_470_2L/1 -> [VeSignalLostCODR_470_2L]
  VeSignalLostDR_213_2L/1 -> [VeSignalLostDR_213_2L]
  From76/1 -> AcsExtAvl/10(VeSignalLost2R_463_2L)
  [VeSignalLost2R_463_2L] -> AcsEntyAvl/10(VeSignalLost2R_463_2L)
  [VeSignalLost3R_46C_2L] -> AcsEntyAvl/12(VeSignalLost3R_46C_2L)
  [VeSignalLost3R_46C_2L] -> VipMdAvl/22(VeSignalLost3R_46C_2L)
  [VeSignalLost3R_46C_2L] -> LugMdAvl/14(VeSignalLost3R_46C_2L)
  [VeSignalLost2R_463_2L] -> RcvyMdAvl/11(VeSignalLost2R_463_2L)
  AcsEntryPosLrnd/1 -> AcsEntyAvl/5(AcsEntryPosLrnd)
  VIPLtPosLrnd/1 -> VipMdAvl/5(VIPLtPosLrnd)
  VIPRtPosLrnd/1 -> VipMdAvl/6(VIPRtPosLrnd)
  LugLtPosLrnd/1 -> LugMdAvl/3(LugLtPosLrnd)
  LugRtPosLrnd/1 -> LugMdAvl/4(LugRtPosLrnd)
  KeSMSbRoofSWEnable/1 -> [KeSMSbRoofSWEnable]
  Ground/1 -> HMIMd8Cfg_2R/1
  Ground1/1 -> HMIMd8Avl_2R/1
  Ground2/1 -> HMIMd9Cfg_2L/1
  Ground3/1 -> HMIMd9Avl_2L/1
  Ground4/1 -> HMIMd10Cfg_2R/1
  Ground5/1 -> HMIMd10Avl_2R/1
  Ground6/1 -> HMIMd11Cfg_2R/1
  Ground7/1 -> HMIMd11Avl_2R/1
  Ground8/1 -> HMIMd12Cfg_2L/1
  Ground9/1 -> HMIMd12Avl_2L/1
  Ground10/1 -> HMIMd13Cfg_2L/1
  Ground11/1 -> HMIMd13Avl_2L/1
  Ground13/1 -> HMIMd14Cfg_2R/1
  Ground15/1 -> HMIMd14Avl_2R/1
  Ground16/1 -> HMIMd15Cfg_2L/1
  Ground18/1 -> HMIMd15Avl_2L/1
  Ground26/1 -> HMIMd6Cfg_2L/1
  Ground28/1 -> HMIMd6Avl_2L/1
  Ground33/1 -> HMIMd7Cfg_2R/1
  Ground35/1 -> HMIMd7Avl_2R/1
  [KeSMSbRoofSWEnable] -> StPassCmprtMdRfCtrlSwCstStAvl/1
  From9/1 -> AcsExtAvl/6(IsDrvStSwAct)
  From14/1 -> AcsExtAvl/7(IsPasStSwAct)
  [Is2RStSwAct] -> VipMdAvl/15(Is2RStSwAct)
  VeSignalLostSDM_195_2L/1 -> "CommCond "/11(VeSignalLostSDM_195_2L)
  From27/1 -> IntimacyMd/1(CommCond)
  From30/1 -> IntimacyMd/2(IntimacyMdConfig)
  From31/1 -> IntimacyMd/3(SecRwLtStPosRclRspStat)
  From42/1 -> IntimacyMd/4(SecRwRtStPosRclRspStat)
  From43/1 -> IntimacyMd/7(Is2LStSwAct)
  From48/1 -> IntimacyMd/8(Is2RStSwAct)
  From49/1 -> IntimacyMd/9(VeSignalLost2R_463_2L)
  From56/1 -> FamilyMd/1(CommCond)
  From57/1 -> FamilyMd/2(FamilyMdConfig)
  From58/1 -> FamilyMd/3(SecRwLtStPosRclRspStat)
  From59/1 -> FamilyMd/4(SecRwRtStPosRclRspStat)
  From61/1 -> FamilyMd/8(Is2RStSwAct)
  From60/1 -> FamilyMd/7(Is2LStSwAct)
  From64/1 -> FamilyMd/10(Is3RStSwAct)
  From90/1 -> FamilyMd/9(Is3LStSwAct)
  From91/1 -> FamilyMd/11(VeSignalLost2R_463_2L)
  From92/1 -> FamilyMd/12(VeSignalLost3L_468_2L)
  From93/1 -> FamilyMd/13(VeSignalLost3R_46C_2L)
  From95/1 -> LyingMd/1(CommCond)
  From94/1 -> LyingMd/2(LyingMdConfig)
  From96/1 -> LyingMd/3(SecRwLtStPosRclRspStat)
  From97/1 -> LyingMd/4(SecRwRtStPosRclRspStat)
  From98/1 -> LyingMd/7(Is2LStSwAct)
  From99/1 -> LyingMd/8(Is2RStSwAct)
  From100/1 -> LyingMd/9(SecRwLtStChldLkReq)
  From101/1 -> LyingMd/10(SecRwRtStChldLkReq)
  From102/1 -> LyingMd/11(VeSignalLost2R_463_2L)
  VeSignalLostFireWall_1D2_2L/1 -> "CommCond "/12(VeSignalLostFireWall_1D2_2L)
  "CommCond "/2("CommCondWithSpeed ") -> [CommCondWithSpeed]
  "CommCond "/7(DiagAbgDly) -> Data Type Conversion/1
  Data Type Conversion/1 -> DiagAbgDly/1
  Data Type Conversion1/1 -> DiagVehMovState/1
  "CommCond "/8(DiagVehMovState) -> Data Type Conversion1/1
  Data Type Conversion2/1 -> DiagVehSpdAvgDrvn/1
  "CommCond "/9(DiagVehSpdAvgDrvn) -> Data Type Conversion2/1
  HMI_2L_StMd1_Config/1 -> [HMI_2L_StMd1_Config], HMIMd1Cfg_2L/1
  HMI_2R_StMd1_Config/1 -> [HMI_2R_StMd1_Config], HMIMd1Cfg_2R/1
  StPassCmprtMdCtrl_Md1_VCUConfig/1 -> [StPassCmprtMdCtrl_Md1_VCUConfig], StPassCmprtMdCtrl_Md1_VCUCfg/1
  StSrv_StMd1_Config/1 -> [StSrv_StMd1_Config], StSrvCfg_Md1/1
  HMI_2L_StMd2_Config/1 -> [HMI_2L_StMd2_Config], HMIMd2Cfg_2L/1
  HMI_2R_StMd2_Config/1 -> [HMI_2R_StMd2_Config], HMIMd2Cfg_2R/1
  StPassCmprtMdCtrl_Md2_VCUConfig/1 -> [StPassCmprtMdCtrl_Md2_VCUConfig], StPassCmprtMdCtrl_Md2_VCUCfg/1
  StSrv_StMd2_Config/1 -> [StSrv_StMd2_Config], StSrvCfg_Md2/1
  HMI_2L_StMd10_Config/1 -> [HMI_2L_StMd10_Config], HMIMd10Cfg_2L/1
  HMI_2R_StMd12_Config/1 -> [HMI_2R_StMd12_Config], HMIMd12Cfg_2R/1
  StSrv_StMd10_Config/1 -> [StSrv_StMd10_Config], StSrvCfg_Md10/1
  StSrv_StMd12_Config/1 -> [StSrv_StMd12_Config], StSrvCfg_Md12/1
  StPassCmprtMdCtrl_Md10_VCUConfig/1 -> [StPassCmprtMdCtrl_Md10_VCUConfig], StPassCmprtMdCtrl_Md10_VCUCfg/1
  StPassCmprtMdCtrl_Md12_VCUConfig/1 -> [StPassCmprtMdCtrl_Md12_VCUConfig], StPassCmprtMdCtrl_Md12_VCUCfg/1
  HMI_2L_StMd4_Config/1 -> [HMI_2L_StMd4_Config], HMIMd4Cfg_2L/1
  HMI_2R_StMd4_Config/1 -> [HMI_2R_StMd4_Config], HMIMd4Cfg_2R/1
  StSrv_StMd4_Config/1 -> [StSrv_StMd4_Config], StSrvCfg_Md4/1
  StPassCmprtMdCtrl_Md4_VCUConfig/1 -> [StPassCmprtMdCtrl_Md4_VCUConfig], StPassCmprtMdCtrl_Md4_VCUCfg/1
  HMI_2L_StMd3_Config/1 -> [HMI_2L_StMd3_Config], HMIMd3Cfg_2L/1
  HMI_2R_StMd3_Config/1 -> [HMI_2R_StMd3_Config], HMIMd3Cfg_2R/1
  StSrv_StMd3_Config/1 -> [StSrv_StMd3_Config], StSrvCfg_Md3/1
  StPassCmprtMdCtrl_Md3_VCUConfig/1 -> [StPassCmprtMdCtrl_Md3_VCUConfig], StPassCmprtMdCtrl_Md3_VCUCfg/1
  HMI_2L_StMd8_Config/1 -> [HMI_2L_StMd8_Config], HMIMd8Cfg_2L/1
  StSrv_StMd8_Config/1 -> [StSrv_StMd8_Config], StSrvCfg_Md8/1
  StPassCmprtMdCtrl_Md8_VCUConfig/1 -> [StPassCmprtMdCtrl_Md8_VCUConfig], StPassCmprtMdCtrl_Md8_VCUCfg/1
  StSrv_StMd9_Config/1 -> [StSrv_StMd9_Config], StSrvCfg_Md9/1
  StPassCmprtMdCtrl_Md9_VCUConfig/1 -> [StPassCmprtMdCtrl_Md9_VCUConfig], StPassCmprtMdCtrl_Md9_VCUCfg/1
  HMI_2L_StMd11_Config/1 -> [HMI_2L_StMd11_Config], HMIMd11Cfg_2L/1
  HMI_2R_StMd13_Config/1 -> [HMI_2R_StMd13_Config], HMIMd13Cfg_2R/1
  StSrv_StMd11_Config/1 -> [StSrv_StMd11_Config], StSrvCfg_Md11/1
  StSrv_StMd13_Config/1 -> [StSrv_StMd13_Config], StSrvCfg_Md13/1
  StPassCmprtMdCtrl_Md11_VCUConfig/1 -> [StPassCmprtMdCtrl_Md11_VCUConfig], StPassCmprtMdCtrl_Md11_VCUCfg/1
  StPassCmprtMdCtrl_Md13_VCUConfig/1 -> [StPassCmprtMdCtrl_Md13_VCUConfig], StPassCmprtMdCtrl_Md13_VCUCfg/1
  HMI_2L_StMd5_Config/1 -> [HMI_2L_StMd5_Config], HMIMd5Cfg_2L/1
  StPassCmprtMdCtrl_Md5_VCUConfig/1 -> [StPassCmprtMdCtrl_Md5_VCUConfig], StPassCmprtMdCtrl_Md5_VCUCfg/1
  StSrv_StMd5_Config/1 -> [StSrv_StMd5_Config], StSrvCfg_Md5/1
  HMI_2R_StMd6_Config/1 -> [HMI_2R_StMd6_Config], HMIMd6Cfg_2R/1
  HMI_2L_StMd7_Config/1 -> [HMI_2L_StMd7_Config], HMIMd7Cfg_2L/1
  StPassCmprtMdCtrl_Md6_VCUConfig/1 -> [StPassCmprtMdCtrl_Md6_VCUConfig], StPassCmprtMdCtrl_Md6_VCUCfg/1
  StSrv_StMd6_Config/1 -> [StSrv_StMd6_Config], StSrvCfg_Md6/1
  StPassCmprtMdCtrl_Md7_VCUConfig/1 -> [StPassCmprtMdCtrl_Md7_VCUConfig], StPassCmprtMdCtrl_Md7_VCUCfg/1
  StSrv_StMd7_Config/1 -> [StSrv_StMd7_Config], StSrvCfg_Md7/1
  HMI_2L_StMd14_Config/1 -> [HMI_2L_StMd14_Config], HMIMd14Cfg_2L/1
  HMI_2R_StMd15_Config/1 -> [HMI_2R_StMd15_Config], HMIMd15Cfg_2R/1
  StPassCmprtMdCtrl_Md14_VCUConfig/1 -> [StPassCmprtMdCtrl_Md14_VCUConfig], StPassCmprtMdCtrl_Md14_VCUCfg/1
  StPassCmprtMdCtrl_Md15_VCUConfig/1 -> [StPassCmprtMdCtrl_Md15_VCUConfig], StPassCmprtMdCtrl_Md15_VCUCfg/1
  StSrv_StMd14_Config/1 -> [StSrv_StMd14_Config], StSrvCfg_Md14/1
  StSrv_StMd15_Config/1 -> [StSrv_StMd15_Config], StSrvCfg_Md15/1
  From105/1 -> LgrstOpenLtMd/2(LgrstLtMdConfig)
  From106/1 -> LgrstOpenLtMd/1(CommCond)
  From107/1 -> LgrstOpenLtMd/3(SecRwLtStPosRclRspStat)
  From109/1 -> LgrstOpenLtMd/6(Is2LStSwAct)
  Ground14/1 -> HMIMd16Cfg_2R/1
  HMI_2L_StMd16_Config/1 -> [HMI_2L_StMd16_Config], HMIMd16Cfg_2L/1
  StPassCmprtMdCtrl_Md16_VCUConfig/1 -> [StPassCmprtMdCtrl_Md16_VCUConfig], StPassCmprtMdCtrl_Md16_VCUCfg/1
  StSrv_StMd16_Config/1 -> [StSrv_StMd16_Config], StSrvCfg_Md16/1
  Ground12/1 -> HMIMd17Cfg_2R/1
  HMI_2L_StMd17_Config/1 -> [HMI_2L_StMd17_Config], HMIMd17Cfg_2L/1
  StPassCmprtMdCtrl_Md17_VCUConfig/1 -> [StPassCmprtMdCtrl_Md17_VCUConfig], StPassCmprtMdCtrl_Md17_VCUCfg/1
  StSrv_StMd17_Config/1 -> [StSrv_StMd17_Config], StSrvCfg_Md17/1
  Ground17/1 -> HMIMd18Cfg_2L/1
  Ground19/1 -> HMIMd19Cfg_2L/1
  StPassCmprtMdCtrl_Md18_VCUConfig/1 -> [StPassCmprtMdCtrl_Md18_VCUConfig], StPassCmprtMdCtrl_Md18_VCUCfg/1
  StSrv_StMd18_Config/1 -> [StSrv_StMd18_Config], StSrvCfg_Md18/1
  HMI_2R_StMd18_Config/1 -> [HMI_2R_StMd18_Config], HMIMd18Cfg_2R/1
  StPassCmprtMdCtrl_Md19_VCUConfig/1 -> [StPassCmprtMdCtrl_Md19_VCUConfig], StPassCmprtMdCtrl_Md19_VCUCfg/1
  HMI_2R_StMd19_Config/1 -> [HMI_2R_StMd19_Config], HMIMd19Cfg_2R/1
  StSrv_StMd19_Config/1 -> [StSrv_StMd19_Config], StSrvCfg_Md19/1
  From116/1 -> LgrstOpenRtMd/6(Is2RStSwAct)
  From115/1 -> LgrstOpenRtMd/3(SecRwRtStPosRclRspStat)
  From108/1 -> LgrstOpenRtMd/2(LgrstRtMdConfig)
  From113/1 -> LgrstOpenRtMd/1(CommCond)
  From121/1 -> LgrstOpenRtMd/7(VeSignalLost2R_463_2L)
  Ground20/1 -> HMIMd5Cfg_2R/1
  HMI_2R_StMd20_Config/1 -> [HMI_2R_StMd20_Config], HMIMd20Cfg_2R/1
  StPassCmprtMdCtrl_Md20_VCUConfig/1 -> [StPassCmprtMdCtrl_Md20_VCUConfig], StPassCmprtMdCtrl_Md20_VCUCfg/1
  StSrv_StMd20_Config/1 -> [StSrv_StMd20_Config], StSrvCfg_Md20/1
  IfVeSMSeStNumConfig/1 -> [IfVeSMSeStNumConfig]
  [IfVeSMSeStNumConfig] -> Equal1/1, Equal/1
  Constant/1 -> Equal/2
  Constant1/1 -> Equal1/2
  Equal/1 -> AND2/1
  Equal1/1 -> AND2/2
  AND2/1 -> Switch/2
  Constant2/1 -> Switch/1
  Constant3/1 -> Switch/3
  Switch/1 -> [WholeVehMemConfig], [Big4SeatMdConfig], [PassReclinerMdConfig], [FamilyMdConfig], [IntimacyMdConfig], [LugMdConfig], [AcsMdExtConfig], [AcsMdEtryConfig]
  [IfVeSMSeStNumConfig] -> Equal3/1, Equal2/1
  Constant5/1 -> Equal2/2
  Constant6/1 -> Equal3/2
  Equal2/1 -> AND3/1
  Equal3/1 -> AND3/2
  AND3/1 -> Switch1/2
  Constant7/1 -> Switch1/1
  Constant8/1 -> Switch1/3
  Switch1/1 -> AND4/1, [LgrstRtMdConfig], [LgrstLtMdConfig], [LyingMdConfig]
  [StPassCmprtMdCtrl_Md1_VCUConfig] -> Switch2/2
  Switch2/1 -> StPassCmprtMdCtrl_Md1_VCUAvl/1
  Switch3/1 -> HMIMd1Avl_2L/1
  [HMI_2L_StMd1_Config] -> Switch3/2
  Constant9/1 -> Switch2/3, Switch3/3, Switch4/3, Switch5/3
  Switch4/1 -> HMIMd1Avl_2R/1
  [HMI_2R_StMd1_Config] -> Switch4/2
  Switch5/1 -> StSrvAvl_Md1/1
  [StSrv_StMd1_Config] -> Switch5/2
  [HMI_2L_StMd4_Config] -> Switch6/2
  Switch6/1 -> HMIMd4Avl_2L/1
  Constant10/1 -> Switch6/3, Switch8/3, Switch9/3, Switch7/3
  Switch7/1 -> HMIMd4Avl_2R/1
  [HMI_2R_StMd4_Config] -> Switch7/2
  Switch8/1 -> StPassCmprtMdCtrl_Md4_VCUAvl/1
  [StPassCmprtMdCtrl_Md4_VCUConfig] -> Switch8/2
  [AcsMdEntyAvl] -> Switch5/1, Switch4/1, Switch3/1, Switch2/1
  Switch9/1 -> StSrvAvl_Md4/1
  [StSrv_StMd4_Config] -> Switch9/2
  [AcsMdExtAvl] -> Switch9/1, Switch8/1, Switch7/1, Switch6/1
  AND/1 -> [VipMdAllAvl]
  [VipMdAllAvl] -> Switch13/1, Switch12/1, Switch11/1, Switch10/1
  [HMI_2R_StMd2_Config] -> Switch10/2
  Constant11/1 -> Switch10/3, Switch13/3, Switch12/3, Switch11/3
  Switch10/1 -> HMIMd2Avl_2R/1
  Switch11/1 -> HMIMd2Avl_2L/1
  [HMI_2L_StMd2_Config] -> Switch11/2
  Switch12/1 -> StPassCmprtMdCtrl_Md2_VCUAvl/1
  [StPassCmprtMdCtrl_Md2_VCUConfig] -> Switch12/2
  Switch13/1 -> StSrvAvl_Md2/1
  [StSrv_StMd2_Config] -> Switch13/2
  [HMI_2L_StMd10_Config] -> Switch14/2
  Constant12/1 -> Switch16/3, Switch15/3, Switch14/3
  [VipMdLtAvl] -> Switch16/1, Switch15/1, Switch14/1
  Switch14/1 -> HMIMd10Avl_2L/1
  Switch15/1 -> StPassCmprtMdCtrl_Md10_VCUAvl/1
  [StPassCmprtMdCtrl_Md10_VCUConfig] -> Switch15/2
  Switch16/1 -> StSrvAvl_Md10/1
  [StSrv_StMd10_Config] -> Switch16/2
  [HMI_2R_StMd12_Config] -> Switch17/2
  [VipMdRtAvl] -> Switch19/1, Switch18/1, Switch17/1
  Constant13/1 -> Switch19/3, Switch18/3, Switch17/3
  Switch17/1 -> HMIMd12Avl_2R/1
  Switch18/1 -> StPassCmprtMdCtrl_Md12_VCUAvl/1
  [StPassCmprtMdCtrl_Md12_VCUConfig] -> Switch18/2
  [StSrv_StMd12_Config] -> Switch19/2
  Switch19/1 -> StSrvAvl_Md12/1
  AND1/1 -> [LugMdAllAvl]
  [HMI_2L_StMd3_Config] -> Switch20/2
  [LugMdAllAvl] -> Switch23/1, Switch22/1, Switch21/1, Switch20/1
  Switch20/1 -> HMIMd3Avl_2L/1
  Constant14/1 -> Switch23/3, Switch22/3, Switch21/3, Switch20/3
  Switch21/1 -> HMIMd3Avl_2R/1
  [HMI_2R_StMd3_Config] -> Switch21/2
  Switch22/1 -> StPassCmprtMdCtrl_Md3_VCUAvl/1
  [StPassCmprtMdCtrl_Md3_VCUConfig] -> Switch22/2
  Switch23/1 -> StSrvAvl_Md3/1
  [StSrv_StMd3_Config] -> Switch23/2
  HMI_2R_StMd9_Config/1 -> [HMI_2R_StMd9_Config], HMIMd9Cfg_2R/1
  Switch24/1 -> HMIMd8Avl_2L/1
  [HMI_2L_StMd8_Config] -> Switch24/2
  [LugMdLtAvl] -> Switch26/1, Switch25/1, Switch24/1
  Constant15/1 -> Switch26/3, Switch25/3, Switch24/3
  [StSrv_StMd8_Config] -> Switch25/2
  Switch25/1 -> StSrvAvl_Md8/1
  Switch26/1 -> StPassCmprtMdCtrl_Md8_VCUAvl/1
  [StPassCmprtMdCtrl_Md8_VCUConfig] -> Switch26/2
  [HMI_2R_StMd9_Config] -> Switch27/2
  [LugMdRtAvl] -> Switch29/1, Switch28/1, Switch27/1
  Constant16/1 -> Switch29/3, Switch28/3, Switch27/3
  Switch27/1 -> HMIMd9Avl_2R/1
  Switch28/1 -> StSrvAvl_Md9/1
  [StSrv_StMd9_Config] -> Switch28/2
  Switch29/1 -> StPassCmprtMdCtrl_Md9_VCUAvl/1
  [StPassCmprtMdCtrl_Md9_VCUConfig] -> Switch29/2
  [RcvyMdLtAvl] -> Switch32/1, Switch31/1, Switch30/1
  [HMI_2L_StMd11_Config] -> Switch30/2
  Constant17/1 -> Switch32/3, Switch31/3, Switch30/3
  Switch30/1 -> HMIMd11Avl_2L/1
  [StSrv_StMd11_Config] -> Switch31/2
  Switch31/1 -> StSrvAvl_Md11/1
  Switch32/1 -> StPassCmprtMdCtrl_Md11_VCUAvl/1
  [StPassCmprtMdCtrl_Md11_VCUConfig] -> Switch32/2
  [HMI_2R_StMd13_Config] -> Switch33/2
  [RcvyMdRtAvl] -> Switch35/1, Switch34/1, Switch33/1
  Constant18/1 -> Switch35/3, Switch34/3, Switch33/3
  Switch33/1 -> HMIMd13Avl_2R/1
  Switch34/1 -> StSrvAvl_Md13/1
  [StSrv_StMd13_Config] -> Switch34/2
  Switch35/1 -> StPassCmprtMdCtrl_Md13_VCUAvl/1
  [StPassCmprtMdCtrl_Md13_VCUConfig] -> Switch35/2
  [HMI_2L_StMd5_Config] -> Switch36/2
  [IntimacyLMdAvl] -> Switch38/1, Switch37/1, Switch36/1
  Switch36/1 -> HMIMd5Avl_2L/1
  Constant19/1 -> Switch38/3, Switch37/3, Switch36/3
  Switch37/1 -> StSrvAvl_Md5/1
  [StSrv_StMd5_Config] -> Switch37/2
  Switch38/1 -> StPassCmprtMdCtrl_Md5_VCUAvl/1
  [StPassCmprtMdCtrl_Md5_VCUConfig] -> Switch38/2
  [HMI_2R_StMd20_Config] -> Switch39/2
  [IntimacyRMdAvl] -> Switch41/1, Switch40/1, Switch39/1
  Switch39/1 -> HMIMd20Avl_2R/1
  Constant20/1 -> Switch41/3, Switch40/3, Switch39/3
  Switch40/1 -> StSrvAvl_Md20/1
  [StSrv_StMd20_Config] -> Switch40/2
  Switch41/1 -> StPassCmprtMdCtrl_Md20_VCUAvl/1
  [StPassCmprtMdCtrl_Md20_VCUConfig] -> Switch41/2
  [HMI_2L_StMd7_Config] -> Switch42/2
  [FamilyMdLtAvl] -> Switch44/1, Switch43/1, Switch42/1
  Switch42/1 -> HMIMd7Avl_2L/1
  Constant21/1 -> Switch44/3, Switch43/3, Switch42/3
  Switch43/1 -> StSrvAvl_Md7/1
  [StSrv_StMd7_Config] -> Switch43/2
  Switch44/1 -> StPassCmprtMdCtrl_Md7_VCUAvl/1
  [StPassCmprtMdCtrl_Md7_VCUConfig] -> Switch44/2
  Switch45/1 -> HMIMd6Avl_2R/1
  [HMI_2R_StMd6_Config] -> Switch45/2
  [FamilyMdRtAvl] -> Switch47/1, Switch46/1, Switch45/1
  Constant22/1 -> Switch47/3, Switch46/3, Switch45/3
  Switch46/1 -> StSrvAvl_Md6/1
  [StSrv_StMd6_Config] -> Switch46/2
  Switch47/1 -> StPassCmprtMdCtrl_Md6_VCUAvl/1
  [StPassCmprtMdCtrl_Md6_VCUConfig] -> Switch47/2
  [HMI_2L_StMd14_Config] -> Switch48/2
  [LyingMdLtAvl] -> Switch50/1, Switch49/1, Switch48/1
  Switch48/1 -> HMIMd14Avl_2L/1
  Constant23/1 -> Switch50/3, Switch49/3, Switch48/3
  Switch49/1 -> StSrvAvl_Md14/1
  [StSrv_StMd14_Config] -> Switch49/2
  Switch50/1 -> StPassCmprtMdCtrl_Md14_VCUAvl/1
  [StPassCmprtMdCtrl_Md14_VCUConfig] -> Switch50/2
  Switch51/1 -> HMIMd15Avl_2R/1
  [HMI_2R_StMd15_Config] -> Switch51/2
  [LyingMdRtAvl] -> Switch53/1, Switch52/1, Switch51/1
  Constant24/1 -> Switch51/3, Switch53/3, Switch52/3
  Switch52/1 -> StSrvAvl_Md15/1
  [StSrv_StMd15_Config] -> Switch52/2
  Switch53/1 -> StPassCmprtMdCtrl_Md15_VCUAvl/1
  [StPassCmprtMdCtrl_Md15_VCUConfig] -> Switch53/2
  Switch54/1 -> HMIMd16Avl_2L/1
  [HMI_2L_StMd16_Config] -> Switch54/2
  [LgrstOpenLtMdAvl] -> Switch56/1, Switch55/1, Switch54/1
  Constant25/1 -> Switch56/3, Switch55/3, Switch54/3
  Switch55/1 -> StSrvAvl_Md16/1
  [StSrv_StMd16_Config] -> Switch55/2
  Switch56/1 -> StPassCmprtMdCtrl_Md16_VCUAvl/1
  [StPassCmprtMdCtrl_Md16_VCUConfig] -> Switch56/2
  [HMI_2L_StMd17_Config] -> Switch57/2
  [LgrstCloseLtMdAvl] -> Switch59/1, Switch58/1, Switch57/1
  Constant26/1 -> Switch59/3, Switch58/3, Switch57/3
  Switch57/1 -> HMIMd17Avl_2L/1
  [StSrv_StMd17_Config] -> Switch58/2
  Switch58/1 -> StSrvAvl_Md17/1
  Switch59/1 -> StPassCmprtMdCtrl_Md17_VCUAvl/1
  [StPassCmprtMdCtrl_Md17_VCUConfig] -> Switch59/2
  Switch60/1 -> HMIMd18Avl_2R/1
  [HMI_2R_StMd18_Config] -> Switch60/2
  [LgrstOpenRtMdAvl] -> Switch60/1, Switch61/1, Switch62/1
  Constant27/1 -> Switch62/3, Switch61/3, Switch60/3
  Switch61/1 -> StSrvAvl_Md18/1
  [StSrv_StMd18_Config] -> Switch61/2
  Switch62/1 -> StPassCmprtMdCtrl_Md18_VCUAvl/1
  [StPassCmprtMdCtrl_Md18_VCUConfig] -> Switch62/2
  [HMI_2R_StMd19_Config] -> Switch63/2
  [LgrstCloseRtMdAvl] -> Switch65/1, Switch64/1, Switch63/1
  Switch63/1 -> HMIMd19Avl_2R/1
  Constant28/1 -> Switch63/3, Switch65/3, Switch64/3
  Switch64/1 -> StSrvAvl_Md19/1
  [StSrv_StMd19_Config] -> Switch64/2
  Switch65/1 -> StPassCmprtMdCtrl_Md19_VCUAvl/1
  [StPassCmprtMdCtrl_Md19_VCUConfig] -> Switch65/2
  [VeSignalLost2R_463_2L] -> LugMdAvl/15(VeSignalLost2R_463_2L)
  KeSMSLegrstDisFwdBkwdPos/1 -> [KeSMSLegrstDisFwdBkwdPos]
  SecRwLtStFrwdBkwdPos/1 -> [SecRwLtStFrwdBkwdPos]
  "SecRwLtStFrwdBkwdPosV "/1 -> Terminator_75/1
  "SecRwRtStFrwdBkwdPos "/1 -> [SecRwRtStFrwdBkwdPos]
  "SecRwRtStFrwdBkwdPosV "/1 -> Terminator_1/1
  From201/1 -> AcsEntry4s2LMd/2(AcsEntry4s2LMdConfig)
  From202/1 -> AcsEntry4s2LMd/1(CommCond)
  From209/1 -> AcsEntry4s2LMd/5(Is2LStSwAct)
  Switch66/1 -> StPassCmprtMdCtrl_Md21_VCUAvl/1
  Switch69/1 -> StSrvAvl_Md21/1
  Constant29/1 -> Switch66/3, Switch69/3, Switch67/3
  [AcsEntry4s2LAvl] -> Switch69/1, Switch67/1, Switch66/1
  [StPassCmprtMdCtrl_Md21_VCUConfig] -> Switch66/2
  Switch67/1 -> HMIMd21Avl_2L/1
  HMI_2L_StMd21_Config/1 -> [HMI_2L_StMd21_Config], HMIMd21Cfg_2L/1
  StPassCmprtMdCtrl_Md21_VCUConfig/1 -> [StPassCmprtMdCtrl_Md21_VCUConfig], StPassCmprtMdCtrl_Md21_VCUCfg/1
  StSrv_StMd21_Config/1 -> [StSrv_StMd21_Config], StSrvCfg_Md21/1
  [StSrv_StMd21_Config] -> Switch69/2
  [HMI_2L_StMd21_Config] -> Switch67/2
  From203/1 -> AcsEntry4s2RMd/1(CommCond)
  From204/1 -> AcsEntry4s2RMd/2(AcsEntry4s2RMdConfig)
  From216/1 -> AcsEntry4s2RMd/5(Is2RStSwAct)
  From217/1 -> AcsEntry4s2RMd/6(VeSignalLost2R_463_2L)
  HMI_2R_StMd23_Config/1 -> [HMI_2R_StMd23_Config], HMIMd23Cfg_2R/1
  StPassCmprtMdCtrl_Md23_VCUConfig/1 -> [StPassCmprtMdCtrl_Md23_VCUConfig], StPassCmprtMdCtrl_Md23_VCUCfg/1
  StSrv_StMd23_Config/1 -> [StSrv_StMd23_Config], StSrvCfg_Md23/1
  [StPassCmprtMdCtrl_Md23_VCUConfig] -> Switch68/2
  [StSrv_StMd23_Config] -> Switch71/2
  [HMI_2R_StMd23_Config] -> Switch70/2
  [AcsEntry4s2RAvl] -> Switch71/1, Switch70/1, Switch68/1
  Constant30/1 -> Switch71/3, Switch70/3, Switch68/3
  Switch68/1 -> StPassCmprtMdCtrl_Md23_VCUAvl/1
  Switch70/1 -> HMIMd23Avl_2R/1
  Switch71/1 -> StSrvAvl_Md23/1
  From205/1 -> AcsExit4s2LMd/2(AcsExit4s2LMdConfig)
  From223/1 -> AcsExit4s2LMd/1(CommCond)
  From224/1 -> AcsExit4s2LMd/5(Is2LStSwAct)
  HMI_2L_StMd22_Config/1 -> [HMI_2L_StMd22_Config], HMIMd22Cfg_2L/1
  StPassCmprtMdCtrl_Md22_VCUConfig/1 -> [StPassCmprtMdCtrl_Md22_VCUConfig], StPassCmprtMdCtrl_Md22_VCUCfg/1
  StSrv_StMd22_Config/1 -> [StSrv_StMd22_Config], StSrvCfg_Md22/1
  [StPassCmprtMdCtrl_Md22_VCUConfig] -> Switch72/2
  [HMI_2L_StMd22_Config] -> Switch73/2
  [StSrv_StMd22_Config] -> Switch74/2
  [AcsExit4s2LAvl] -> Switch72/1, Switch74/1, Switch73/1
  Constant31/1 -> Switch72/3, Switch74/3, Switch73/3
  Switch72/1 -> StPassCmprtMdCtrl_Md22_VCUAvl/1
  Switch73/1 -> HMIMd22Avl_2L/1
  Switch74/1 -> StSrvAvl_Md22/1
  From208/1 -> AcsExit4s2RMd/2(AcsExit4s2RMdConfig)
  From229/1 -> AcsExit4s2RMd/1(CommCond)
  From231/1 -> AcsExit4s2RMd/5(Is2RStSwAct)
  From232/1 -> AcsExit4s2RMd/6(VeSignalLost2R_463_2L)
  HMI_2R_StMd24_Config/1 -> [HMI_2R_StMd24_Config], HMIMd24Cfg_2R/1
  StPassCmprtMdCtrl_Md24_VCUConfig/1 -> [StPassCmprtMdCtrl_Md24_VCUConfig], StPassCmprtMdCtrl_Md24_VCUCfg/1
  StSrv_StMd24_Config/1 -> [StSrv_StMd24_Config], StSrvCfg_Md24/1
  [StPassCmprtMdCtrl_Md24_VCUConfig] -> Switch75/2
  [HMI_2R_StMd24_Config] -> Switch76/2
  [StSrv_StMd24_Config] -> Switch77/2
  [AcsExit4s2RAvl] -> Switch77/1, Switch76/1, Switch75/1
  Constant32/1 -> Switch77/3, Switch76/3, Switch75/3
  Switch75/1 -> StPassCmprtMdCtrl_Md24_VCUAvl/1
  Switch76/1 -> HMIMd24Avl_2R/1
  Switch77/1 -> StSrvAvl_Md24/1
  From215/1 -> AcsEntryAll4sFwdMd/2(AcsEntryAll4sFwdMdConfig)
  From206/1 -> AcsEntry4s2LMd/3(SecRwLtStChldLkReq)
  From237/1 -> AcsEntry4s2RMd/3(SecRwRtStChldLkReq)
  From207/1 -> AcsExit4s2LMd/3(SecRwLtStChldLkReq)
  From222/1 -> AcsExit4s2RMd/3(SecRwRtStChldLkReq)
  From230/1 -> AcsEntryAll4sFwdMd/1(CommCond)
  From239/1 -> AcsEntryAll4sFwdMd/3(SecRwLtStChldLkReq)
  From238/1 -> AcsEntryAll4sFwdMd/4(SecRwRtStChldLkReq)
  From240/1 -> AcsEntryAll4sFwdMd/7(Is2RStSwAct)
  From241/1 -> AcsEntryAll4sFwdMd/6(Is2LStSwAct)
  From242/1 -> AcsEntryAll4sFwdMd/8(VeSignalLost2R_463_2L)
  HMI_2L_StMd26_Config/1 -> [HMI_2L_StMd26_Config], HMIMd26Cfg_2L/1
  HMI_2R_StMd26_Config/1 -> [HMI_2R_StMd26_Config], HMIMd26Cfg_2R/1
  StPassCmprtMdCtrl_Md26_VCUConfig/1 -> [StPassCmprtMdCtrl_Md26_VCUConfig], StPassCmprtMdCtrl_Md26_VCUCfg/1
  StSrv_StMd26_Config/1 -> [StSrv_StMd26_Config], StSrvCfg_Md26/1
  [HMI_2L_StMd26_Config] -> Switch78/2
  [AcsEntryAll4sFwdAvl] -> Switch81/1, Switch80/1, Switch79/1, Switch78/1
  [HMI_2R_StMd26_Config] -> Switch79/2
  [StSrv_StMd26_Config] -> Switch81/2
  Constant33/1 -> Switch81/3, Switch80/3, Switch79/3, Switch78/3
  Switch78/1 -> HMIMd26Avl_2L/1
  Switch79/1 -> HMIMd26Avl_2R/1
  Switch80/1 -> StPassCmprtMdCtrl_Md26_VCUAvl/1
  Switch81/1 -> StSrvAvl_Md26/1
  From214/1 -> AcsEntryAll4sBwdMd/2(AcsEntryAll4sBwdMdConfig)
  From248/1 -> AcsEntryAll4sBwdMd/1(CommCond)
  From249/1 -> AcsEntryAll4sBwdMd/3(SecRwLtStChldLkReq)
  From250/1 -> AcsEntryAll4sBwdMd/4(SecRwRtStChldLkReq)
  From251/1 -> AcsEntryAll4sBwdMd/6(Is2LStSwAct)
  From252/1 -> AcsEntryAll4sBwdMd/7(Is2RStSwAct)
  From253/1 -> AcsEntryAll4sBwdMd/8(VeSignalLost2R_463_2L)
  HMI_2L_StMd25_Config/1 -> [HMI_2L_StMd25_Config], HMIMd25Cfg_2L/1
  HMI_2R_StMd25_Config/1 -> [HMI_2R_StMd25_Config], HMIMd25Cfg_2R/1
  StPassCmprtMdCtrl_Md25_VCUConfig/1 -> [StPassCmprtMdCtrl_Md25_VCUConfig], StPassCmprtMdCtrl_Md25_VCUCfg/1
  StSrv_StMd25_Config/1 -> [StSrv_StMd25_Config], StSrvCfg_Md25/1
  [HMI_2L_StMd25_Config] -> Switch82/2
  [HMI_2R_StMd25_Config] -> Switch83/2
  [StSrv_StMd25_Config] -> Switch85/2
  [AcsEntryAll4sBwdAvl] -> Switch85/1, Switch84/1, Switch83/1, Switch82/1
  Constant34/1 -> Switch85/3, Switch84/3, Switch83/3, Switch82/3
  Switch82/1 -> HMIMd25Avl_2L/1
  Switch83/1 -> HMIMd25Avl_2R/1
  Switch84/1 -> StPassCmprtMdCtrl_Md25_VCUAvl/1
  Switch85/1 -> StSrvAvl_Md25/1
  IfKeSMSbSeatMovFrwdBkwdEnable/1 -> Equal4/1
  Constant35/1 -> Equal4/2
  Equal4/1 -> AND4/2
  AND4/1 -> [AcsEntryAll4sFwdMdConfig], [AcsEntryAll4sBwdMdConfig], [AcsExit4s2RMdConfig], [AcsExit4s2LMdConfig], [AcsEntry4s2RMdConfig], [AcsEntry4s2LMdConfig]
  [StPassCmprtMdCtrl_Md26_VCUConfig] -> Terminator_2/1
  Constant36/1 -> Switch80/2
  [StPassCmprtMdCtrl_Md25_VCUConfig] -> Terminator_3/1
  Constant37/1 -> Switch84/2
  PasReclinerMd/1("PasReclinerAvl ") -> [PasReclinerAvl], "PasReclinerAvl "/1
  [CommCond] -> PasReclinerMd/1(CommCond)
  [PassReclinerMdConfig] -> PasReclinerMd/2(PassReclinerMdConfig)
  PassReclinerPosLrnd/1 -> PasReclinerMd/3(PassReclinerPosLrnd)
  [IsPasStSwAct] -> PasReclinerMd/5(IsPasStSwAct)
  [StPassCmprtMdCtrl_Md30_VCUConfig] -> Switch86/2
  [PasReclinerAvl] -> Switch87/1, Switch86/1
  Constant38/1 -> Switch87/3, Switch86/3
  [VeSignalLostCODR_470_2L] -> PasReclinerMd/7(VeSignalLostCODR_470_2L)
  StPassCmprtMdCtrl_Md30_VCUConfig/1 -> [StPassCmprtMdCtrl_Md30_VCUConfig], StPassCmprtMdCtrl_Md30_VCUCfg/1
  StSrv_StMd30_Config/1 -> [StSrv_StMd30_Config], StSrvCfg_Md30/1
  StPassCmprtMdCtrl_Md31_VCUConfig/1 -> [StPassCmprtMdCtrl_Md31_VCUConfig], StPassCmprtMdCtrl_Md31_VCUCfg/1
  StSrv_StMd31_Config/1 -> [StSrv_StMd31_Config], StSrvCfg_Md31/1
  Switch86/1 -> StPassCmprtMdCtrl_Md30_VCUAvl/1
  [StSrv_StMd30_Config] -> Switch87/2
  Switch87/1 -> StSrvAvl_Md30/1
  [StPassCmprtMdCtrl_Md31_VCUConfig] -> Switch88/2
  Constant39/1 -> Switch89/3, Switch88/3
  [PasReclinerExitAvl] -> Switch89/1, Switch88/1
  Switch88/1 -> StPassCmprtMdCtrl_Md31_VCUAvl/1
  [StSrv_StMd31_Config] -> Switch89/2
  Switch89/1 -> StSrvAvl_Md31/1
  [CommCond] -> unfoldMd/1(CommCond)
  unfold3LPosLrnd/1 -> unfoldMd/3(unfold3LPosLrnd)
  unfoldMd/1("unfold3LAvl ") -> unfold3LAvl/1, [unfold3LAvl]
  StPassCmprtMdCtrl_Md32_VCUConfig/1 -> [StPassCmprtMdCtrl_Md32_VCUConfig], StPassCmprtMdCtrl_Md32_VCUCfg/1
  StSrv_StMd32_Config/1 -> [StSrv_StMd32_Config], StSrvCfg_Md32/1
  [StPassCmprtMdCtrl_Md32_VCUConfig] -> Switch90/2
  [unfold3LAvl] -> Switch91/1, Switch90/1
  Constant40/1 -> Switch90/3, Switch91/3
  [StSrv_StMd32_Config] -> Switch91/2
  Switch90/1 -> StPassCmprtMdCtrl_Md32_VCUAvl/1
  Switch91/1 -> StSrvAvl_Md32/1
  [unfoldMdConfig] -> unfoldMd/2(unfoldMdConfig)
  unfoldMd/2("unfold3RAvl ") -> unfold3RAvl/1, [unfold3RAvl]
  unfold3RPosLrnd/1 -> unfoldMd/4(unfold3RPosLrnd)
  [ThdRwLtStOccStat] -> unfoldMd/5(ThdRwLtStOccStat)
  [ThdRwCtStOccStat] -> unfoldMd/6(ThdRwCtStOccStat)
  [ThdRwRtStOccStat] -> unfoldMd/7(ThdRwRtStOccStat)
  [Is2LStSwAct] -> unfoldMd/8(Is2LStSwAct)
  [Is3LStSwAct] -> unfoldMd/10(Is3LStSwAct)
  [Is3RStSwAct] -> unfoldMd/11(Is3RStSwAct)
  [Is2RStSwAct] -> unfoldMd/9(Is2RStSwAct)
  [VeSignalLost3R_46C_2L] -> unfoldMd/14(VeSignalLost3R_46C_2L)
  [VeSignalLost2R_463_2L] -> unfoldMd/12(VeSignalLost2R_463_2L)
  [IfVeSMSeStNumConfig] -> unfoldMd/15(IfVeSMSeStNumConfig)
  [SecRwLtStPosRclRspStat] -> unfoldMd/16(SecRwLtStPosRclRspStat)
  [SecRwRtStPosRclRspStat] -> unfoldMd/17(SecRwRtStPosRclRspStat)
  Constant4/1 -> [VipMdConfig], [RcvyMdConfig]
  AND5/1 -> [VipAllOutMdAvl]
  VIPRtOutPosLrnd/1 -> VipOutMdAvl/6(VIPRtOutPosLrnd)
  VIPLtOutPosLrnd/1 -> VipOutMdAvl/5(VIPLtOutPosLrnd)
  [IfVeSMSeStNumConfig] -> VipOutMdAvl/15(IfVeSMSeStNumConfig)
  [SecRwRtStPosRclRspStat] -> VipOutMdAvl/4(SecRwRtStPosRclRspStat)
  [SecRwLtStPosRclRspStat] -> VipOutMdAvl/3(SecRwLtStPosRclRspStat)
  [VipMdConfig] -> VipOutMdAvl/2(VipMdConfig)
  VipOutMdAvl/2(VipRtOutMdAvl) -> VipRtOutMdAvl/1, [VipRtOutMdAvl], AND5/2
  [CommCond] -> VipOutMdAvl/1(CommCond)
  VipOutMdAvl/1(VipLtOutMdAvl) -> AND5/1, [VipLtOutMdAvl], VipLtOutMdAvl/1
  [SecRwRtStChldLkReq] -> VipOutMdAvl/8(SecRwRtStChldLkReq)
  [SecRwLtStChldLkReq] -> VipOutMdAvl/7(SecRwLtStChldLkReq)
  [Is2LStSwAct] -> VipOutMdAvl/11(Is2LStSwAct)
  [Is2RStSwAct] -> VipOutMdAvl/12(Is2RStSwAct)
  [Is3LStSwAct] -> VipOutMdAvl/13(Is3LStSwAct)
  [Is3RStSwAct] -> VipOutMdAvl/14(Is3RStSwAct)
  [VeSignalLost2R_463_2L] -> VipOutMdAvl/17(VeSignalLost2R_463_2L)
  [VeSignalLost3R_46C_2L] -> VipOutMdAvl/19(VeSignalLost3R_46C_2L)
  [IsPasStSwAct] -> VipOutMdAvl/10(IsPasStSwAct)
  [StSrv_StMd29_Config] -> Switch95/2
  [VipRtOutMdAvl] -> Switch101/1, Switch100/1
  [StPassCmprtMdCtrl_Md27_VCUConfig] -> Switch97/2
  [StSrv_StMd27_Config] -> Switch98/2
  [VipLtOutMdAvl] -> Switch98/1, Switch97/1
  Switch98/1 -> StSrvAvl_Md27/1
  Constant43/1 -> Switch101/3, Switch100/3
  Switch100/1 -> StPassCmprtMdCtrl_Md28_VCUAvl/1
  Switch95/1 -> StSrvAvl_Md29/1
  Constant42/1 -> Switch98/3, Switch97/3
  [StPassCmprtMdCtrl_Md29_VCUConfig] -> Switch94/2
  Switch101/1 -> StSrvAvl_Md28/1
  Constant41/1 -> Switch94/3, Switch95/3
  [VipAllOutMdAvl] -> Switch95/1, Switch94/1
  Switch94/1 -> StPassCmprtMdCtrl_Md29_VCUAvl/1
  [StPassCmprtMdCtrl_Md28_VCUConfig] -> Switch100/2
  [StSrv_StMd28_Config] -> Switch101/2
  Switch97/1 -> StPassCmprtMdCtrl_Md27_VCUAvl/1
  StPassCmprtMdCtrl_Md27_VCUConfig/1 -> [StPassCmprtMdCtrl_Md27_VCUConfig], StPassCmprtMdCtrl_Md27_VCUCfg/1
  StSrv_StMd27_Config/1 -> [StSrv_StMd27_Config], StSrvCfg_Md27/1
  StPassCmprtMdCtrl_Md28_VCUConfig/1 -> [StPassCmprtMdCtrl_Md28_VCUConfig], StPassCmprtMdCtrl_Md28_VCUCfg/1
  StSrv_StMd28_Config/1 -> [StSrv_StMd28_Config], StSrvCfg_Md28/1
  StSrv_StMd29_Config/1 -> [StSrv_StMd29_Config], StSrvCfg_Md29/1
  StPassCmprtMdCtrl_Md29_VCUConfig/1 -> [StPassCmprtMdCtrl_Md29_VCUConfig], StPassCmprtMdCtrl_Md29_VCUCfg/1
  [VeSignalLostCODR_470_2L] -> VipOutMdAvl/16(VeSignalLostCODR_470_2L)
  [Is2LStSwAct] -> LugMdAvl/10(Is2LStSwAct)
  [Is2RStSwAct] -> LugMdAvl/11(Is2RStSwAct)
  From17/1 -> AcsEntry4s2LMd/6(SecRwLtStPosRclRspStat)
  From18/1 -> AcsEntry4s2RMd/7(SecRwRtStPosRclRspStat)
  From53/1 -> AcsExit4s2LMd/6(SecRwLtStPosRclRspStat)
  From277/1 -> AcsExit4s2RMd/7(SecRwRtStPosRclRspStat)
  From278/1 -> AcsEntryAll4sFwdMd/9(SecRwLtStPosRclRspStat)
  From279/1 -> AcsEntryAll4sFwdMd/10(SecRwRtStPosRclRspStat)
  From295/1 -> AcsEntryAll4sBwdMd/9(SecRwLtStPosRclRspStat)
  From296/1 -> AcsEntryAll4sBwdMd/10(SecRwRtStPosRclRspStat)
  [IsPasStSwAct] -> VipMdAvl/13(IsPasStSwAct)
  [VeSignalLostCODR_470_2L] -> VipMdAvl/20(VeSignalLostCODR_470_2L)
  ThdRwLtStCshnFldUpwdDnwdPos/1 -> [ThdRwLtStCshnFldUpwdDnwdPos]
  ThdRwLtStCshnFldUpwdDnwdPosV/1 -> [ThdRwLtStCshnFldUpwdDnwdPosV]
  ThdRwRtStCshnFldUpwdDnwdPos/1 -> [ThdRwRtStCshnFldUpwdDnwdPos]
  ThdRwRtStCshnFldUpwdDnwdPosV/1 -> [ThdRwRtStCshnFldUpwdDnwdPosV]
  [ThdRwLtStCshnFldUpwdDnwdPos] -> VipMdAvl/23(ThdRwLtStCshnFldUpwdDnwdPos)
  [ThdRwLtStCshnFldUpwdDnwdPosV] -> VipMdAvl/24(ThdRwLtStCshnFldUpwdDnwdPosV)
  [ThdRwRtStCshnFldUpwdDnwdPos] -> VipMdAvl/25(ThdRwRtStCshnFldUpwdDnwdPos)
  [ThdRwRtStCshnFldUpwdDnwdPosV] -> VipMdAvl/26(ThdRwRtStCshnFldUpwdDnwdPosV)
  ThdRwLtStChldLkReq/1 -> [ThdRwLtStChldLkReq]
  [ThdRwLtStChldLkReq] -> VipOutMdAvl/9(ThdRwLtStChldLkReq)
  [ThdRwLtStCshnFldUpwdDnwdPos] -> VipOutMdAvl/20(ThdRwLtStCshnFldUpwdDnwdPos)
  [ThdRwLtStCshnFldUpwdDnwdPosV] -> VipOutMdAvl/21(ThdRwLtStCshnFldUpwdDnwdPosV)
  [ThdRwRtStCshnFldUpwdDnwdPos] -> VipOutMdAvl/22(ThdRwRtStCshnFldUpwdDnwdPos)
  [ThdRwRtStCshnFldUpwdDnwdPosV] -> VipOutMdAvl/23(ThdRwRtStCshnFldUpwdDnwdPosV)
  [ThdRwLtStChldLkReq] -> VipMdAvl/12(ThdRwLtStChldLkReq)
  AcsExitPosLrnd/1 -> Terminator_4/1
  Ground21/1 -> [AcsMdExtAvl], AcsMdExtAvl/1
  IntimacyLPosLrnd/1 -> Terminator_5/1
  Ground22/1 -> [IntimacyLMdAvl], IntimacyLMdAvl/1
  IntimacyRPosLrnd/1 -> Terminator_6/1
  Ground23/1 -> [IntimacyRMdAvl], IntimacyRMdAvl/1
  FamilyLtPosLrnd/1 -> Terminator_7/1
  FamilyRtPosLrnd/1 -> Terminator_8/1
  Ground24/1 -> FamilyMdLtAvl/1, [FamilyMdLtAvl]
  Ground25/1 -> FamilyMdRtAvl/1, [FamilyMdRtAvl]
  LyingLtPosLrnd/1 -> Terminator_9/1
  LyingRtPosLrnd/1 -> Terminator_10/1
  Ground27/1 -> LyingMdLtAvl/1, [LyingMdLtAvl]
  Ground29/1 -> LyingMdRtAvl/1, [LyingMdRtAvl]
  LgrstOpenLtPosLrnd/1 -> Terminator_11/1
  LgrstCloseLtPosLrnd/1 -> Terminator_12/1
  Ground30/1 -> LgrstOpenLtMdAvl/1, [LgrstOpenLtMdAvl]
  Ground31/1 -> LgrstCloseLtMdAvl/1, [LgrstCloseLtMdAvl]
  LgrstOpenRtPosLrnd/1 -> Terminator_13/1
  LgrstCloseRtPosLrnd/1 -> Terminator_14/1
  Ground32/1 -> LgrstOpenRtMdAvl/1, [LgrstOpenRtMdAvl]
  Ground34/1 -> LgrstCloseRtMdAvl/1, [LgrstCloseRtMdAvl]
  AcsEntry4s2LPosLrnd/1 -> Terminator_15/1
  Ground36/1 -> AcsEntry4s2LAvl/1, [AcsEntry4s2LAvl]
  AcsEntry4s2RPosLrnd/1 -> Terminator_16/1
  Ground37/1 -> AcsEntry4s2RAvl/1, [AcsEntry4s2RAvl]
  AcsExit4s2LPosLrnd/1 -> Terminator_17/1
  Ground38/1 -> AcsExit4s2LAvl/1, [AcsExit4s2LAvl]
  AcsExit4s2RPosLrnd/1 -> Terminator_18/1
  Ground39/1 -> AcsExit4s2RAvl/1, [AcsExit4s2RAvl]
  AcsEntryAll4sFwdPosLrnd/1 -> Terminator_19/1
  Ground40/1 -> AcsEntryAll4sFwdAvl/1, [AcsEntryAll4sFwdAvl]
  Ground41/1 -> AcsEntryAll4sBwdAvl/1, [AcsEntryAll4sBwdAvl]
  AcsEntryAll4sBwdPosLrnd/1 -> Terminator_20/1
  [IfVeSMSeStNumConfig] -> AcsEntyAvl/13(IfVeSMSeStNumConfig)
  NotSecRowLeStOccStatBDFSrc/1 -> AcsEntyAvl/14(NotSecRowLeStOccStatBDFSrc)
  NotSecRowRtStOccStatBDFSrc/1 -> AcsEntyAvl/15(NotSecRowRtStOccStatBDFSrc)
  [ThdRwLtStOccStat] -> AcsEntyAvl/16(ThdRwLtStOccStat)
  [ThdRwCtStOccStat] -> AcsEntyAvl/17(ThdRwCtStOccStat)
  [ThdRwRtStOccStat] -> AcsEntyAvl/18(ThdRwRtStOccStat)
  PasReclinerMd/2(PasReclinerExitAvl) -> [PasReclinerExitAvl], PasReclinerExitAvl/1
  [SecRwLtStChldLkReq] -> LugMdAvl/21(SecRwLtStChldLkReq)
  [SecRwRtStChldLkReq] -> LugMdAvl/22(SecRwRtStChldLkReq)
  [ThdRwLtStChldLkReq] -> LugMdAvl/23(ThdRwLtStChldLkReq)
  LugMdAvl/1(LugMdLtAvl) -> [LugMdLtAvl], AND1/1, LugMdLtAvl/1
  StPassCmprtMdCtrl_Md53_VCUConfig/1 -> [StPassCmprtMdCtrl_Md53_VCUConfig], StPassCmprtMdCtrl_Md53_VCUCfg/1
  [StPassCmprtMdCtrl_Md53_VCUConfig] -> Switch92/2
  [unfold3RAvl] -> Switch92/1
  Constant44/1 -> Switch92/3
  Switch92/1 -> StPassCmprtMdCtrl_Md53_VCUAvl/1
  SecRwLtStBkReclnUpwdDnwdPos/1 -> [SecRwLtStBkReclnUpwdDnwdPos]
  SecRwLtStBkReclnUpwdDnwdPosV/1 -> [SecRwLtStBkReclnUpwdDnwdPosV]
  SecRwRtStBkReclnUpwdDnwdPos/1 -> [SecRwRtStBkReclnUpwdDnwdPos]
  SecRwRtStBkReclnUpwdDnwdPosV/1 -> [SecRwRtStBkReclnUpwdDnwdPosV]
  KeSMSuSecRwStBackPosDelta/1 -> [KeSMSuSecRwStBackPosDelta]
  [SecRwLtStBkReclnUpwdDnwdPos] -> LugMdAvl/16(SecRwLtStBkReclnUpwdDnwdPos)
  [SecRwLtStBkReclnUpwdDnwdPosV] -> LugMdAvl/17(SecRwLtStBkReclnUpwdDnwdPosV)
  [SecRwRtStBkReclnUpwdDnwdPos] -> LugMdAvl/18(SecRwRtStBkReclnUpwdDnwdPos)
  [SecRwRtStBkReclnUpwdDnwdPosV] -> LugMdAvl/19(SecRwRtStBkReclnUpwdDnwdPosV)
  [KeSMSuSecRwStBackPosDelta] -> LugMdAvl/20(KeSMSuSecRwStBackPosDelta)
  [SecRwLtStBkReclnUpwdDnwdPos] -> unfoldMd/18(SecRwLtStBkReclnUpwdDnwdPos)
  [SecRwLtStBkReclnUpwdDnwdPosV] -> unfoldMd/19(SecRwLtStBkReclnUpwdDnwdPosV)
  [SecRwRtStBkReclnUpwdDnwdPos] -> unfoldMd/20(SecRwRtStBkReclnUpwdDnwdPos)
  [SecRwRtStBkReclnUpwdDnwdPosV] -> unfoldMd/21(SecRwRtStBkReclnUpwdDnwdPosV)
  [KeSMSuSecRwStBackPosDelta] -> unfoldMd/25(KeSMSuSecRwStBackPosDelta)
  [ThdRwLtStChldLkReq] -> unfoldMd/22(ThdRwLtStChldLkReq)
  [SecRwLtStChldLkReq] -> unfoldMd/23(SecRwLtStChldLkReq)
  [SecRwRtStChldLkReq] -> unfoldMd/24(SecRwRtStChldLkReq)
  VeSignalLost3L_468_2L/1 -> [VeSignalLost3L_468_2L]
  [VeSignalLost3L_468_2L] -> AcsEntyAvl/11(VeSignalLost3L_468_2L)
  [Is3LStSwAct] -> AcsEntyAvl/8(Is3LStSwAct)
  [VeSignalLost2R_463_2L] -> VipMdAvl/19("VeSignalLost2R_463_2L ")
  [VeSignalLost3L_468_2L] -> VipMdAvl/21(VeSignalLost3L_468_2L)
  [VeSignalLost3L_468_2L] -> LugMdAvl/13(VeSignalLost3L_468_2L)
  [VeSignalLost3L_468_2L] -> unfoldMd/13(VeSignalLost3L_468_2L)
  [VeSignalLost3L_468_2L] -> VipOutMdAvl/18(VeSignalLost3L_468_2L)
  StPassCmprtMdCtrl_Md56_VCUConfig/1 -> [StPassCmprtMdCtrl_Md56_VCUConfig], StPassCmprtMdCtrl_Md56_VCUCfg/1
  [StPassCmprtMdCtrl_Md56_VCUConfig] -> Switch93/2
  Constant45/1 -> Switch93/3
  Switch93/1 -> StPassCmprtMdCtrl_Md56_VCUAvl/1
  Constant46/1 -> Equal5/2
  [IfVeSMSeStNumConfig] -> Equal5/1
  Constant48/1 -> Switch96/3
  Constant47/1 -> Switch96/1
  Equal5/1 -> Switch96/2
  Switch96/1 -> [unfoldMdConfig]
  KeSMSuThrdRwCushFoldPosThreshold/1 -> [KeSMSuThrdRwCushFoldPosThreshold]
  [KeSMSuThrdRwCushFoldPosThreshold] -> VipOutMdAvl/24(KeSMSuThrdRwCushFoldPosThreshold)
  [KeSMSuThrdRwCushFoldPosThreshold] -> VipMdAvl/27(KeSMSuThrdRwCushFoldPosThreshold)
  [SecRwLtStPosRclRspStat] -> LugMdAvl/24(SecRwLtStPosRclRspStat)
  [SecRwRtStPosRclRspStat] -> LugMdAvl/25(SecRwRtStPosRclRspStat)
  StPassCmprtMdCtrl_Md57_VCUConfig/1 -> [StPassCmprtMdCtrl_Md57_VCUConfig], StPassCmprtMdCtrl_Md57_VCUCfg/1
  StPassCmprtMdCtrl_Md58_VCUConfig/1 -> [StPassCmprtMdCtrl_Md58_VCUConfig], StPassCmprtMdCtrl_Md58_VCUCfg/1
  [StPassCmprtMdCtrl_Md57_VCUConfig] -> Switch99/2
  [VipMdRtAvl] -> Switch99/1
  Constant49/1 -> Switch99/3
  Switch99/1 -> StPassCmprtMdCtrl_Md57_VCUAvl/1
  [StPassCmprtMdCtrl_Md58_VCUConfig] -> Switch102/2
  Constant50/1 -> Switch102/3
  [VipRtOutMdAvl] -> Switch102/1
  Switch102/1 -> StPassCmprtMdCtrl_Md58_VCUAvl/1
  PasReclinerPosAvail/1 -> PasReclinerMd/9(PasReclinerPosAvail)
  [Big4SeatMdConfig] -> AcsEntyAvl/19(Big4SeatMdConfig)
  AcsEntyAvl/2(Big4SeatAvl) -> [Big4SeatAvl], Big4SeatAvl/1
  [Big4SeatAvl] -> Switch93/1
  KeSMSwAcsMd32SecRwLtStBkReclnUpwdDnwdPos1/1 -> [KeSMSwAcsMd32SecRwLtStBkReclnUpwdDnwdPos1]
  KeSMSwAcsMd53SecRwRtStBkReclnUpwdDnwdPos1/1 -> [KeSMSwAcsMd53SecRwRtStBkReclnUpwdDnwdPos1]
  [KeSMSwAcsMd32SecRwLtStBkReclnUpwdDnwdPos1] -> unfoldMd/26(KeSMSwAcsMd32SecRwLtStBkReclnUpwdDnwdPos1)
  [KeSMSwAcsMd53SecRwRtStBkReclnUpwdDnwdPos1] -> unfoldMd/27(KeSMSwAcsMd53SecRwRtStBkReclnUpwdDnwdPos1)
  [KeSMSwAcsMd8SecRwLtStBkReclnUpwdDnwdPos] -> LugMdAvl/26(KeSMSwAcsMd8SecRwLtStBkReclnUpwdDnwdPos)
  [KeSMSwAcsMd9SecRwRtStBkReclnUpwdDnwdPos] -> LugMdAvl/27(KeSMSwAcsMd9SecRwRtStBkReclnUpwdDnwdPos)
  KeSMSwAcsMd8SecRwLtStBkReclnUpwdDnwdPos/1 -> [KeSMSwAcsMd8SecRwLtStBkReclnUpwdDnwdPos]
  KeSMSwAcsMd9SecRwRtStBkReclnUpwdDnwdPos/1 -> [KeSMSwAcsMd9SecRwRtStBkReclnUpwdDnwdPos]
  [PassStPosRclRspStat] -> VipMdAvl/28(PassStPosRclRspStat)
  [PassStPosRclRspStat] -> PasReclinerMd/10(PassStPosRclRspStat)
  [PassStPosRclRspStat] -> VipOutMdAvl/25(PassStPosRclRspStat)
  NotCoDrvStOccStatBDFSrc/1 -> [NotCoDrvStOccStatBDFSrc]
  [NotCoDrvStOccStatBDFSrc] -> PasReclinerMd/4(NotCoDrvStOccStatBDFSrc)
  [Is2RStSwAct] -> PasReclinerMd/6(Is2RStSwAct)
  [VeSignalLost2R_463_2L] -> PasReclinerMd/8(VeSignalLost2R_463_2L)
  [CommCondWithSpeed] -> WholeVehMem/1(CommCondWithSpeed)
  [WholeVehMemConfig] -> WholeVehMem/2(WholeVehMemConfig)
  [SecRwLtStPosRclRspStat] -> WholeVehMem/4(SecRwLtStPosRclRspStat)
  [SecRwRtStPosRclRspStat] -> WholeVehMem/5(SecRwRtStPosRclRspStat)
  [PassStPosRclRspStat] -> WholeVehMem/3(PassStPosRclRspStat)
  WholeVehMemPosLrnd/1 -> WholeVehMem/6(WholeVehMemPosLrnd)
  [IsPasStSwAct] -> WholeVehMem/7(IsPasStSwAct)
  [Is2LStSwAct] -> WholeVehMem/8(Is2LStSwAct)
  [Is2RStSwAct] -> WholeVehMem/9(Is2RStSwAct)
  [Is3LStSwAct] -> WholeVehMem/10(Is3LStSwAct)
  [Is3RStSwAct] -> WholeVehMem/11(Is3RStSwAct)
  [VeSignalLostCODR_470_2L] -> WholeVehMem/12(VeSignalLostCODR_470_2L)
  [VeSignalLost2R_463_2L] -> WholeVehMem/13(VeSignalLost2R_463_2L)
  [VeSignalLost3L_468_2L] -> WholeVehMem/14(VeSignalLost3L_468_2L)
  [VeSignalLost3R_46C_2L] -> WholeVehMem/15(VeSignalLost3R_46C_2L)
  [SecRwLtStChldLkReq] -> WholeVehMem/16(SecRwLtStChldLkReq)
  [SecRwRtStChldLkReq] -> WholeVehMem/17(SecRwRtStChldLkReq)
  [ThdRwLtStChldLkReq] -> WholeVehMem/18(ThdRwLtStChldLkReq)
  [M61WholeVehMemAvl] -> Switch103/1
  Constant51/1 -> Switch103/3
  Switch103/1 -> StPassCmprtMdCtrl_Md61_VCUAvl/1
  Constant52/1 -> Switch104/3
  [M62WholeVehMemAvl] -> Switch104/1
  Switch104/1 -> StPassCmprtMdCtrl_Md62_VCUAvl/1
  [NotCoDrvStOccStatBDFSrc] -> WholeVehMem/19(NotCoDrvStOccStatBDFSrc)
  [ThdRwLtStOccStat] -> WholeVehMem/20(ThdRwLtStOccStat)
  [ThdRwCtStOccStat] -> WholeVehMem/21(ThdRwCtStOccStat)
  [ThdRwRtStOccStat] -> WholeVehMem/22(ThdRwRtStOccStat)
  KeSMSwSeatBkLimitPos/1 -> WholeVehMem/23(KeSMSwSeatBkLimitPos)
  KeSMSwSeatBkLimitPosDelt/1 -> WholeVehMem/24(KeSMSwSeatBkLimitPosDelt)
  Md61PassStBkReclnTrgtPos/1 -> WholeVehMem/25(Md61PassStBkReclnTrgtPos)
  Md61ThdRwLtStCshnFldUpwdDnwdTrgtPos/1 -> WholeVehMem/26(Md61ThdRwLtStCshnFldUpwdDnwdTrgtPos)
  Md61ThdRwRtStCshnFldUpwdDnwdTrgtPos/1 -> WholeVehMem/27(Md61ThdRwRtStCshnFldUpwdDnwdTrgtPos)
  Md62PassStBkReclnTrgtPos/1 -> WholeVehMem/28(Md62PassStBkReclnTrgtPos)
  Md62ThdRwLtStCshnFldUpwdDnwdTrgtPos/1 -> WholeVehMem/29(Md62ThdRwLtStCshnFldUpwdDnwdTrgtPos)
  Md62ThdRwRtStCshnFldUpwdDnwdTrgtPos/1 -> WholeVehMem/30(Md62ThdRwRtStCshnFldUpwdDnwdTrgtPos)
  KeSMSuThrdRwCushFoldPosDelta/1 -> WholeVehMem/31(KeSMSuThrdRwCushFoldPosDelta)
  WholeVehMem/1(M61WholeVehMemAvl) -> M61WholeVehMemAvl/1, [M61WholeVehMemAvl]
  WholeVehMem/2(M62WholeVehMemAvl) -> M62WholeVehMemAvl/1, [M62WholeVehMemAvl]
  [IfVeSMSeStNumConfig] -> WholeVehMem/32(IfVeSMSeStNumConfig)
  StPassCmprtMdCtrl_Md61_VCUConfig/1 -> [StPassCmprtMdCtrl_Md61_VCUConfig], StPassCmprtMdCtrl_Md61_VCUCfg/1
  StPassCmprtMdCtrl_Md62_VCUConfig/1 -> [StPassCmprtMdCtrl_Md62_VCUConfig], StPassCmprtMdCtrl_Md62_VCUCfg/1
  [StPassCmprtMdCtrl_Md61_VCUConfig] -> Switch103/2
  [StPassCmprtMdCtrl_Md62_VCUConfig] -> Switch104/2
  SysPwrMd/1 -> "CommCond "/1(SysPwrMd)
